simulink model "w3_warplab_trigger_proc"  (Simulink 7.7)
settings: Solver=ode45  StartTime=0.0  StopTime=60  RelTol=1e-3
InitFcn:
  | w3_warplab_trigger_proc_init
StartFcn:
  | w3_warplab_trigger_proc_init
undefined symbols (not defined in the file or in its folder): gcbh, xlBlockLoadCallback, xlGetNormalizedPeriod
libraries: xbsIndex_r4 x1289, xbsEDKLib_r4 x1, simulink x1
(part 3 of 10)

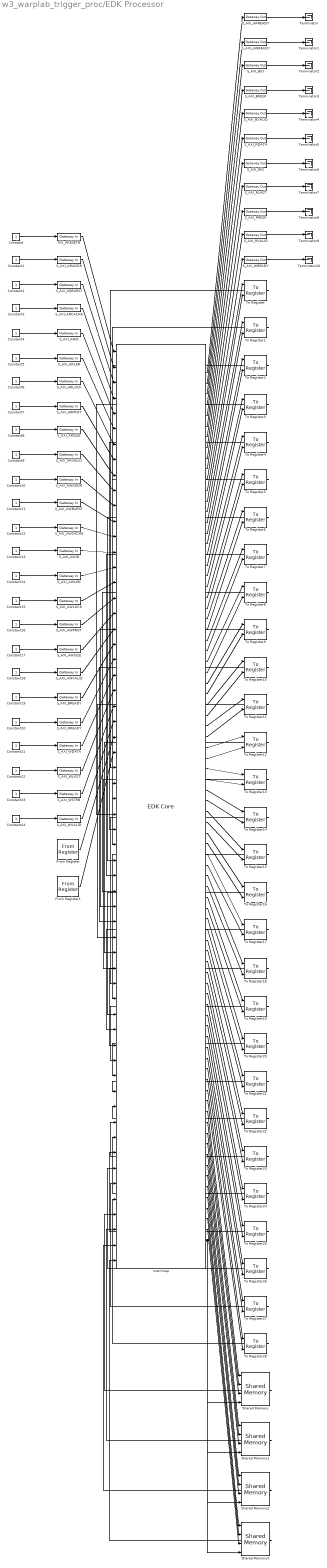
== system w3_warplab_trigger_proc/EDK Processor ==
  AXI_ARESETN : xbsIndex_r4/Gateway In  gui_display_data_type=Fixed-point  arith_type=Boolean  n_bits=16  bin_pt=14  preci_type=Single  exp_width=8  frac_width=24  quantization="Round  (unbiased: +/- Inf)"  overflow=Saturate  period=xlGetNormalizedPeriod()  dbl_ovrd=off  timing_constraint=None  locs_specified=off  LOCs={}  UseAsADC=off  ADCChannel='1'  inherit_from_input=off  hdl_port=on  block_type=gatewayin
  Constant{,1..24} (25 alike) : Constant
  From Register : xbsIndex_r4/From Register  shared_memory_name='CORE_INFO'  init=0  period=xlGetNormalizedPeriod()  ownership=Owned and initialized elsewhere  gui_display_data_type=Fixed-point  arith_type=Unsigned  n_bits=24  bin_pt=0  preci_type=Single  dbl_ovrd=off  block_type=fromreg
      settings: AttributesFormatString=<< %<shared_memory_name> >>  infoedit="Register block that reads data to a shared memory register.  Delay of one sample period."
  From Register1 : xbsIndex_r4/From Register  shared_memory_name='TRIG_OUT'  init=0  period=xlGetNormalizedPeriod()  ownership=Owned and initialized elsewhere  gui_display_data_type=Fixed-point  arith_type=Unsigned  n_bits=6  bin_pt=0  preci_type=Single  dbl_ovrd=off  block_type=fromreg
      settings: AttributesFormatString=<< %<shared_memory_name> >>  infoedit="Register block that reads data to a shared memory register.  Delay of one sample period."
  S_AXI_ARADDR : xbsIndex_r4/Gateway In  gui_display_data_type=Fixed-point  arith_type=Unsigned  n_bits=32  bin_pt=0  preci_type=Single  exp_width=8  frac_width=24  quantization="Round  (unbiased: +/- Inf)"  overflow=Saturate  period=xlGetNormalizedPeriod()  dbl_ovrd=off  timing_constraint=None  locs_specified=off  LOCs={}  UseAsADC=off  ADCChannel='1'  inherit_from_input=off  hdl_port=on  block_type=gatewayin
  S_AXI_ARBURST : xbsIndex_r4/Gateway In  gui_display_data_type=Fixed-point  arith_type=Unsigned  n_bits=2  bin_pt=0  preci_type=Single  exp_width=8  frac_width=24  quantization="Round  (unbiased: +/- Inf)"  overflow=Saturate  period=xlGetNormalizedPeriod()  dbl_ovrd=off  timing_constraint=None  locs_specified=off  LOCs={}  UseAsADC=off  ADCChannel='1'  inherit_from_input=off  hdl_port=on  block_type=gatewayin
  S_AXI_ARCACHE : xbsIndex_r4/Gateway In  gui_display_data_type=Fixed-point  arith_type=Unsigned  n_bits=4  bin_pt=0  preci_type=Single  exp_width=8  frac_width=24  quantization="Round  (unbiased: +/- Inf)"  overflow=Saturate  period=xlGetNormalizedPeriod()  dbl_ovrd=off  timing_constraint=None  locs_specified=off  LOCs={}  UseAsADC=off  ADCChannel='1'  inherit_from_input=off  hdl_port=on  block_type=gatewayin
  S_AXI_ARID : xbsIndex_r4/Gateway In  gui_display_data_type=Fixed-point  arith_type=Unsigned  n_bits=8  bin_pt=0  preci_type=Single  exp_width=8  frac_width=24  quantization="Round  (unbiased: +/- Inf)"  overflow=Saturate  period=xlGetNormalizedPeriod()  dbl_ovrd=off  timing_constraint=None  locs_specified=off  LOCs={}  UseAsADC=off  ADCChannel='1'  inherit_from_input=off  hdl_port=on  block_type=gatewayin
  S_AXI_ARLEN : xbsIndex_r4/Gateway In  gui_display_data_type=Fixed-point  arith_type=Unsigned  n_bits=8  bin_pt=0  preci_type=Single  exp_width=8  frac_width=24  quantization="Round  (unbiased: +/- Inf)"  overflow=Saturate  period=xlGetNormalizedPeriod()  dbl_ovrd=off  timing_constraint=None  locs_specified=off  LOCs={}  UseAsADC=off  ADCChannel='1'  inherit_from_input=off  hdl_port=on  block_type=gatewayin
  S_AXI_ARLOCK : xbsIndex_r4/Gateway In  gui_display_data_type=Fixed-point  arith_type=Unsigned  n_bits=2  bin_pt=0  preci_type=Single  exp_width=8  frac_width=24  quantization="Round  (unbiased: +/- Inf)"  overflow=Saturate  period=xlGetNormalizedPeriod()  dbl_ovrd=off  timing_constraint=None  locs_specified=off  LOCs={}  UseAsADC=off  ADCChannel='1'  inherit_from_input=off  hdl_port=on  block_type=gatewayin
  S_AXI_ARPROT : xbsIndex_r4/Gateway In  gui_display_data_type=Fixed-point  arith_type=Unsigned  n_bits=3  bin_pt=0  preci_type=Single  exp_width=8  frac_width=24  quantization="Round  (unbiased: +/- Inf)"  overflow=Saturate  period=xlGetNormalizedPeriod()  dbl_ovrd=off  timing_constraint=None  locs_specified=off  LOCs={}  UseAsADC=off  ADCChannel='1'  inherit_from_input=off  hdl_port=on  block_type=gatewayin
  S_AXI_ARREADY : xbsIndex_r4/Gateway Out  inherit_from_input=off  hdl_port=on  timing_constraint=None  locs_specified=off  LOCs={}  UseAsDAC=off  DACChannel='1'  block_type=gatewayout
  S_AXI_ARSIZE : xbsIndex_r4/Gateway In  gui_display_data_type=Fixed-point  arith_type=Unsigned  n_bits=3  bin_pt=0  preci_type=Single  exp_width=8  frac_width=24  quantization="Round  (unbiased: +/- Inf)"  overflow=Saturate  period=xlGetNormalizedPeriod()  dbl_ovrd=off  timing_constraint=None  locs_specified=off  LOCs={}  UseAsADC=off  ADCChannel='1'  inherit_from_input=off  hdl_port=on  block_type=gatewayin
  S_AXI_ARVALID : xbsIndex_r4/Gateway In  gui_display_data_type=Fixed-point  arith_type=Boolean  n_bits=16  bin_pt=14  preci_type=Single  exp_width=8  frac_width=24  quantization="Round  (unbiased: +/- Inf)"  overflow=Saturate  period=xlGetNormalizedPeriod()  dbl_ovrd=off  timing_constraint=None  locs_specified=off  LOCs={}  UseAsADC=off  ADCChannel='1'  inherit_from_input=off  hdl_port=on  block_type=gatewayin
  S_AXI_AWADDR : xbsIndex_r4/Gateway In  gui_display_data_type=Fixed-point  arith_type=Unsigned  n_bits=32  bin_pt=0  preci_type=Single  exp_width=8  frac_width=24  quantization="Round  (unbiased: +/- Inf)"  overflow=Saturate  period=xlGetNormalizedPeriod()  dbl_ovrd=off  timing_constraint=None  locs_specified=off  LOCs={}  UseAsADC=off  ADCChannel='1'  inherit_from_input=off  hdl_port=on  block_type=gatewayin
  S_AXI_AWBURST : xbsIndex_r4/Gateway In  gui_display_data_type=Fixed-point  arith_type=Unsigned  n_bits=2  bin_pt=0  preci_type=Single  exp_width=8  frac_width=24  quantization="Round  (unbiased: +/- Inf)"  overflow=Saturate  period=xlGetNormalizedPeriod()  dbl_ovrd=off  timing_constraint=None  locs_specified=off  LOCs={}  UseAsADC=off  ADCChannel='1'  inherit_from_input=off  hdl_port=on  block_type=gatewayin
  S_AXI_AWCACHE : xbsIndex_r4/Gateway In  gui_display_data_type=Fixed-point  arith_type=Unsigned  n_bits=4  bin_pt=0  preci_type=Single  exp_width=8  frac_width=24  quantization="Round  (unbiased: +/- Inf)"  overflow=Saturate  period=xlGetNormalizedPeriod()  dbl_ovrd=off  timing_constraint=None  locs_specified=off  LOCs={}  UseAsADC=off  ADCChannel='1'  inherit_from_input=off  hdl_port=on  block_type=gatewayin
  S_AXI_AWID : xbsIndex_r4/Gateway In  gui_display_data_type=Fixed-point  arith_type=Unsigned  n_bits=8  bin_pt=0  preci_type=Single  exp_width=8  frac_width=24  quantization="Round  (unbiased: +/- Inf)"  overflow=Saturate  period=xlGetNormalizedPeriod()  dbl_ovrd=off  timing_constraint=None  locs_specified=off  LOCs={}  UseAsADC=off  ADCChannel='1'  inherit_from_input=off  hdl_port=on  block_type=gatewayin
  S_AXI_AWLEN : xbsIndex_r4/Gateway In  gui_display_data_type=Fixed-point  arith_type=Unsigned  n_bits=8  bin_pt=0  preci_type=Single  exp_width=8  frac_width=24  quantization="Round  (unbiased: +/- Inf)"  overflow=Saturate  period=xlGetNormalizedPeriod()  dbl_ovrd=off  timing_constraint=None  locs_specified=off  LOCs={}  UseAsADC=off  ADCChannel='1'  inherit_from_input=off  hdl_port=on  block_type=gatewayin
  S_AXI_AWLOCK : xbsIndex_r4/Gateway In  gui_display_data_type=Fixed-point  arith_type=Unsigned  n_bits=2  bin_pt=0  preci_type=Single  exp_width=8  frac_width=24  quantization="Round  (unbiased: +/- Inf)"  overflow=Saturate  period=xlGetNormalizedPeriod()  dbl_ovrd=off  timing_constraint=None  locs_specified=off  LOCs={}  UseAsADC=off  ADCChannel='1'  inherit_from_input=off  hdl_port=on  block_type=gatewayin
  S_AXI_AWPROT : xbsIndex_r4/Gateway In  gui_display_data_type=Fixed-point  arith_type=Unsigned  n_bits=3  bin_pt=0  preci_type=Single  exp_width=8  frac_width=24  quantization="Round  (unbiased: +/- Inf)"  overflow=Saturate  period=xlGetNormalizedPeriod()  dbl_ovrd=off  timing_constraint=None  locs_specified=off  LOCs={}  UseAsADC=off  ADCChannel='1'  inherit_from_input=off  hdl_port=on  block_type=gatewayin
  S_AXI_AWREADY : xbsIndex_r4/Gateway Out  inherit_from_input=off  hdl_port=on  timing_constraint=None  locs_specified=off  LOCs={}  UseAsDAC=off  DACChannel='1'  block_type=gatewayout
  S_AXI_AWSIZE : xbsIndex_r4/Gateway In  gui_display_data_type=Fixed-point  arith_type=Unsigned  n_bits=3  bin_pt=0  preci_type=Single  exp_width=8  frac_width=24  quantization="Round  (unbiased: +/- Inf)"  overflow=Saturate  period=xlGetNormalizedPeriod()  dbl_ovrd=off  timing_constraint=None  locs_specified=off  LOCs={}  UseAsADC=off  ADCChannel='1'  inherit_from_input=off  hdl_port=on  block_type=gatewayin
  S_AXI_AWVALID : xbsIndex_r4/Gateway In  gui_display_data_type=Fixed-point  arith_type=Boolean  n_bits=16  bin_pt=14  preci_type=Single  exp_width=8  frac_width=24  quantization="Round  (unbiased: +/- Inf)"  overflow=Saturate  period=xlGetNormalizedPeriod()  dbl_ovrd=off  timing_constraint=None  locs_specified=off  LOCs={}  UseAsADC=off  ADCChannel='1'  inherit_from_input=off  hdl_port=on  block_type=gatewayin
  S_AXI_BID : xbsIndex_r4/Gateway Out  inherit_from_input=off  hdl_port=on  timing_constraint=None  locs_specified=off  LOCs={}  UseAsDAC=off  DACChannel='1'  block_type=gatewayout
  S_AXI_BREADY : xbsIndex_r4/Gateway In  gui_display_data_type=Fixed-point  arith_type=Boolean  n_bits=16  bin_pt=14  preci_type=Single  exp_width=8  frac_width=24  quantization="Round  (unbiased: +/- Inf)"  overflow=Saturate  period=xlGetNormalizedPeriod()  dbl_ovrd=off  timing_constraint=None  locs_specified=off  LOCs={}  UseAsADC=off  ADCChannel='1'  inherit_from_input=off  hdl_port=on  block_type=gatewayin
  S_AXI_BRESP : xbsIndex_r4/Gateway Out  inherit_from_input=off  hdl_port=on  timing_constraint=None  locs_specified=off  LOCs={}  UseAsDAC=off  DACChannel='1'  block_type=gatewayout
  S_AXI_BVALID : xbsIndex_r4/Gateway Out  inherit_from_input=off  hdl_port=on  timing_constraint=None  locs_specified=off  LOCs={}  UseAsDAC=off  DACChannel='1'  block_type=gatewayout
  S_AXI_RDATA : xbsIndex_r4/Gateway Out  inherit_from_input=off  hdl_port=on  timing_constraint=None  locs_specified=off  LOCs={}  UseAsDAC=off  DACChannel='1'  block_type=gatewayout
  S_AXI_RID : xbsIndex_r4/Gateway Out  inherit_from_input=off  hdl_port=on  timing_constraint=None  locs_specified=off  LOCs={}  UseAsDAC=off  DACChannel='1'  block_type=gatewayout
  S_AXI_RLAST : xbsIndex_r4/Gateway Out  inherit_from_input=off  hdl_port=on  timing_constraint=None  locs_specified=off  LOCs={}  UseAsDAC=off  DACChannel='1'  block_type=gatewayout
  S_AXI_RREADY : xbsIndex_r4/Gateway In  gui_display_data_type=Fixed-point  arith_type=Boolean  n_bits=16  bin_pt=14  preci_type=Single  exp_width=8  frac_width=24  quantization="Round  (unbiased: +/- Inf)"  overflow=Saturate  period=xlGetNormalizedPeriod()  dbl_ovrd=off  timing_constraint=None  locs_specified=off  LOCs={}  UseAsADC=off  ADCChannel='1'  inherit_from_input=off  hdl_port=on  block_type=gatewayin
  S_AXI_RRESP : xbsIndex_r4/Gateway Out  inherit_from_input=off  hdl_port=on  timing_constraint=None  locs_specified=off  LOCs={}  UseAsDAC=off  DACChannel='1'  block_type=gatewayout
  S_AXI_RVALID : xbsIndex_r4/Gateway Out  inherit_from_input=off  hdl_port=on  timing_constraint=None  locs_specified=off  LOCs={}  UseAsDAC=off  DACChannel='1'  block_type=gatewayout
  S_AXI_WDATA : xbsIndex_r4/Gateway In  gui_display_data_type=Fixed-point  arith_type=Unsigned  n_bits=32  bin_pt=0  preci_type=Single  exp_width=8  frac_width=24  quantization="Round  (unbiased: +/- Inf)"  overflow=Saturate  period=xlGetNormalizedPeriod()  dbl_ovrd=off  timing_constraint=None  locs_specified=off  LOCs={}  UseAsADC=off  ADCChannel='1'  inherit_from_input=off  hdl_port=on  block_type=gatewayin
  S_AXI_WLAST : xbsIndex_r4/Gateway In  gui_display_data_type=Fixed-point  arith_type=Boolean  n_bits=16  bin_pt=14  preci_type=Single  exp_width=8  frac_width=24  quantization="Round  (unbiased: +/- Inf)"  overflow=Saturate  period=xlGetNormalizedPeriod()  dbl_ovrd=off  timing_constraint=None  locs_specified=off  LOCs={}  UseAsADC=off  ADCChannel='1'  inherit_from_input=off  hdl_port=on  block_type=gatewayin
  S_AXI_WREADY : xbsIndex_r4/Gateway Out  inherit_from_input=off  hdl_port=on  timing_constraint=None  locs_specified=off  LOCs={}  UseAsDAC=off  DACChannel='1'  block_type=gatewayout
  S_AXI_WSTRB : xbsIndex_r4/Gateway In  gui_display_data_type=Fixed-point  arith_type=Unsigned  n_bits=4  bin_pt=0  preci_type=Single  exp_width=8  frac_width=24  quantization="Round  (unbiased: +/- Inf)"  overflow=Saturate  period=xlGetNormalizedPeriod()  dbl_ovrd=off  timing_constraint=None  locs_specified=off  LOCs={}  UseAsADC=off  ADCChannel='1'  inherit_from_input=off  hdl_port=on  block_type=gatewayin
  S_AXI_WVALID : xbsIndex_r4/Gateway In  gui_display_data_type=Fixed-point  arith_type=Boolean  n_bits=16  bin_pt=14  preci_type=Single  exp_width=8  frac_width=24  quantization="Round  (unbiased: +/- Inf)"  overflow=Saturate  period=xlGetNormalizedPeriod()  dbl_ovrd=off  timing_constraint=None  locs_specified=off  LOCs={}  UseAsADC=off  ADCChannel='1'  inherit_from_input=off  hdl_port=on  block_type=gatewayin
  Shared Memory : xbsIndex_r4/Shared Memory  shared_memory_name='PktOps1'  depth=64  ownership=Owned and Initialized Elsewhere  initVector=sin(pi*(0:15)/16)  en=on  mutex=Unprotected  mode=Read and Write  write_mode=Read Before Write  time_out=0  latency=1  explicit_data_type=off  gui_display_data_type=Fixed-point  arith_type=Unsigned  n_bits=32  bin_pt=0  preci_type=Single  implementation=Block RAM  use_rpm=off  block_type=shmem
      settings: AttributesFormatString=<< %<shared_memory_name> >>
  Shared Memory1 : xbsIndex_r4/Shared Memory  shared_memory_name='PktTemplate1'  depth=64  ownership=Owned and Initialized Elsewhere  initVector=sin(pi*(0:15)/16)  en=on  mutex=Unprotected  mode=Read and Write  write_mode=Read Before Write  time_out=0  latency=1  explicit_data_type=off  gui_display_data_type=Fixed-point  arith_type=Unsigned  n_bits=32  bin_pt=0  preci_type=Single  implementation=Block RAM  use_rpm=off  block_type=shmem
      settings: AttributesFormatString=<< %<shared_memory_name> >>
  Shared Memory2 : xbsIndex_r4/Shared Memory  shared_memory_name='PktOps0'  depth=64  ownership=Owned and Initialized Elsewhere  initVector=sin(pi*(0:15)/16)  en=on  mutex=Unprotected  mode=Read and Write  write_mode=Read Before Write  time_out=0  latency=1  explicit_data_type=off  gui_display_data_type=Fixed-point  arith_type=Unsigned  n_bits=32  bin_pt=0  preci_type=Single  implementation=Block RAM  use_rpm=off  block_type=shmem
      settings: AttributesFormatString=<< %<shared_memory_name> >>
  Shared Memory3 : xbsIndex_r4/Shared Memory  shared_memory_name='PktTemplate0'  depth=64  ownership=Owned and Initialized Elsewhere  initVector=sin(pi*(0:15)/16)  en=on  mutex=Unprotected  mode=Read and Write  write_mode=Read Before Write  time_out=0  latency=1  explicit_data_type=off  gui_display_data_type=Fixed-point  arith_type=Unsigned  n_bits=32  bin_pt=0  preci_type=Single  implementation=Block RAM  use_rpm=off  block_type=shmem
      settings: AttributesFormatString=<< %<shared_memory_name> >>
  Terminator{,1..10} (11 alike) : Terminator
  To Register : xbsIndex_r4/To Register  shared_memory_name='TRIG_ODELAY_CFG_CMPLL'  init=0  ownership=Owned and initialized elsewhere  explicit_data_type=on  gui_display_data_type=Fixed-point  arith_type=Unsigned  n_bits=32  bin_pt=0  preci_type=Single  dbl_ovrd=off  block_type=toreg
      settings: AttributesFormatString=<< %<shared_memory_name> >>  infoedit="Register block that writes data to a shared memory register.  Delay of one sample period."
  To Register1 : xbsIndex_r4/To Register  shared_memory_name='TRIG_IDELAY_CFG_CMPLL'  init=0  ownership=Owned and initialized elsewhere  explicit_data_type=on  gui_display_data_type=Fixed-point  arith_type=Unsigned  n_bits=32  bin_pt=0  preci_type=Single  dbl_ovrd=off  block_type=toreg
      settings: AttributesFormatString=<< %<shared_memory_name> >>  infoedit="Register block that writes data to a shared memory register.  Delay of one sample period."
  To Register10 : xbsIndex_r4/To Register  shared_memory_name='TRIG_IN_CONF_2'  init=0  ownership=Owned and initialized elsewhere  explicit_data_type=on  gui_display_data_type=Fixed-point  arith_type=Unsigned  n_bits=32  bin_pt=0  preci_type=Single  dbl_ovrd=off  block_type=toreg
      settings: AttributesFormatString=<< %<shared_memory_name> >>  infoedit="Register block that writes data to a shared memory register.  Delay of one sample period."
  To Register11 : xbsIndex_r4/To Register  shared_memory_name='TRIG_IN_CONF_0'  init=0  ownership=Owned and initialized elsewhere  explicit_data_type=on  gui_display_data_type=Fixed-point  arith_type=Unsigned  n_bits=32  bin_pt=0  preci_type=Single  dbl_ovrd=off  block_type=toreg
      settings: AttributesFormatString=<< %<shared_memory_name> >>  infoedit="Register block that writes data to a shared memory register.  Delay of one sample period."
  To Register12 : xbsIndex_r4/To Register  shared_memory_name='TRIG_IN_CONF_8'  init=0  ownership=Owned and initialized elsewhere  explicit_data_type=on  gui_display_data_type=Fixed-point  arith_type=Unsigned  n_bits=32  bin_pt=0  preci_type=Single  dbl_ovrd=off  block_type=toreg
      settings: AttributesFormatString=<< %<shared_memory_name> >>  infoedit="Register block that writes data to a shared memory register.  Delay of one sample period."
  To Register13 : xbsIndex_r4/To Register  shared_memory_name='TRIG_IN_CONF_7'  init=0  ownership=Owned and initialized elsewhere  explicit_data_type=on  gui_display_data_type=Fixed-point  arith_type=Unsigned  n_bits=32  bin_pt=0  preci_type=Single  dbl_ovrd=off  block_type=toreg
      settings: AttributesFormatString=<< %<shared_memory_name> >>  infoedit="Register block that writes data to a shared memory register.  Delay of one sample period."
  To Register14 : xbsIndex_r4/To Register  shared_memory_name='TRIG_OUT_5_CONF_0'  init=0  ownership=Owned and initialized elsewhere  explicit_data_type=on  gui_display_data_type=Fixed-point  arith_type=Unsigned  n_bits=32  bin_pt=0  preci_type=Single  dbl_ovrd=off  block_type=toreg
      settings: AttributesFormatString=<< %<shared_memory_name> >>  infoedit="Register block that writes data to a shared memory register.  Delay of one sample period."
  To Register15 : xbsIndex_r4/To Register  shared_memory_name='TRIG_OUT_5_CONF_1'  init=0  ownership=Owned and initialized elsewhere  explicit_data_type=on  gui_display_data_type=Fixed-point  arith_type=Unsigned  n_bits=32  bin_pt=0  preci_type=Single  dbl_ovrd=off  block_type=toreg
      settings: AttributesFormatString=<< %<shared_memory_name> >>  infoedit="Register block that writes data to a shared memory register.  Delay of one sample period."
  To Register16 : xbsIndex_r4/To Register  shared_memory_name='TRIG_OUT_4_CONF_0'  init=0  ownership=Owned and initialized elsewhere  explicit_data_type=on  gui_display_data_type=Fixed-point  arith_type=Unsigned  n_bits=32  bin_pt=0  preci_type=Single  dbl_ovrd=off  block_type=toreg
      settings: AttributesFormatString=<< %<shared_memory_name> >>  infoedit="Register block that writes data to a shared memory register.  Delay of one sample period."
  To Register17 : xbsIndex_r4/To Register  shared_memory_name='TRIG_OUT_0_CONF_0'  init=0  ownership=Owned and initialized elsewhere  explicit_data_type=on  gui_display_data_type=Fixed-point  arith_type=Unsigned  n_bits=32  bin_pt=0  preci_type=Single  dbl_ovrd=off  block_type=toreg
      settings: AttributesFormatString=<< %<shared_memory_name> >>  infoedit="Register block that writes data to a shared memory register.  Delay of one sample period."
  To Register18 : xbsIndex_r4/To Register  shared_memory_name='TRIG_OUT_4_CONF_1'  init=0  ownership=Owned and initialized elsewhere  explicit_data_type=on  gui_display_data_type=Fixed-point  arith_type=Unsigned  n_bits=32  bin_pt=0  preci_type=Single  dbl_ovrd=off  block_type=toreg
      settings: AttributesFormatString=<< %<shared_memory_name> >>  infoedit="Register block that writes data to a shared memory register.  Delay of one sample period."
  To Register19 : xbsIndex_r4/To Register  shared_memory_name='TRIG_OUT_3_CONF_0'  init=0  ownership=Owned and initialized elsewhere  explicit_data_type=on  gui_display_data_type=Fixed-point  arith_type=Unsigned  n_bits=32  bin_pt=0  preci_type=Single  dbl_ovrd=off  block_type=toreg
      settings: AttributesFormatString=<< %<shared_memory_name> >>  infoedit="Register block that writes data to a shared memory register.  Delay of one sample period."
  To Register2 : xbsIndex_r4/To Register  shared_memory_name='TRIG_ODELAY_CFG_DEBUG_HDR'  init=0  ownership=Owned and initialized elsewhere  explicit_data_type=on  gui_display_data_type=Fixed-point  arith_type=Unsigned  n_bits=32  bin_pt=0  preci_type=Single  dbl_ovrd=off  block_type=toreg
      settings: AttributesFormatString=<< %<shared_memory_name> >>  infoedit="Register block that writes data to a shared memory register.  Delay of one sample period."
  To Register20 : xbsIndex_r4/To Register  shared_memory_name='TRIG_OUT_3_CONF_1'  init=0  ownership=Owned and initialized elsewhere  explicit_data_type=on  gui_display_data_type=Fixed-point  arith_type=Unsigned  n_bits=32  bin_pt=0  preci_type=Single  dbl_ovrd=off  block_type=toreg
      settings: AttributesFormatString=<< %<shared_memory_name> >>  infoedit="Register block that writes data to a shared memory register.  Delay of one sample period."
  To Register21 : xbsIndex_r4/To Register  shared_memory_name='TRIG_OUT_2_CONF_0'  init=0  ownership=Owned and initialized elsewhere  explicit_data_type=on  gui_display_data_type=Fixed-point  arith_type=Unsigned  n_bits=32  bin_pt=0  preci_type=Single  dbl_ovrd=off  block_type=toreg
      settings: AttributesFormatString=<< %<shared_memory_name> >>  infoedit="Register block that writes data to a shared memory register.  Delay of one sample period."
  To Register22 : xbsIndex_r4/To Register  shared_memory_name='TRIG_OUT_2_CONF_1'  init=0  ownership=Owned and initialized elsewhere  explicit_data_type=on  gui_display_data_type=Fixed-point  arith_type=Unsigned  n_bits=32  bin_pt=0  preci_type=Single  dbl_ovrd=off  block_type=toreg
      settings: AttributesFormatString=<< %<shared_memory_name> >>  infoedit="Register block that writes data to a shared memory register.  Delay of one sample period."
  To Register23 : xbsIndex_r4/To Register  shared_memory_name='TRIG_OUT_1_CONF_0'  init=0  ownership=Owned and initialized elsewhere  explicit_data_type=on  gui_display_data_type=Fixed-point  arith_type=Unsigned  n_bits=32  bin_pt=0  preci_type=Single  dbl_ovrd=off  block_type=toreg
      settings: AttributesFormatString=<< %<shared_memory_name> >>  infoedit="Register block that writes data to a shared memory register.  Delay of one sample period."
  To Register24 : xbsIndex_r4/To Register  shared_memory_name='TRIG_OUT_1_CONF_1'  init=0  ownership=Owned and initialized elsewhere  explicit_data_type=on  gui_display_data_type=Fixed-point  arith_type=Unsigned  n_bits=32  bin_pt=0  preci_type=Single  dbl_ovrd=off  block_type=toreg
      settings: AttributesFormatString=<< %<shared_memory_name> >>  infoedit="Register block that writes data to a shared memory register.  Delay of one sample period."
  To Register25 : xbsIndex_r4/To Register  shared_memory_name='TRIG_OUT_0_CONF_1'  init=0  ownership=Owned and initialized elsewhere  explicit_data_type=on  gui_display_data_type=Fixed-point  arith_type=Unsigned  n_bits=32  bin_pt=0  preci_type=Single  dbl_ovrd=off  block_type=toreg
      settings: AttributesFormatString=<< %<shared_memory_name> >>  infoedit="Register block that writes data to a shared memory register.  Delay of one sample period."
  To Register26 : xbsIndex_r4/To Register  shared_memory_name='RSSI_PKT_DET_DURATIONS'  init=0  ownership=Owned and initialized elsewhere  explicit_data_type=on  gui_display_data_type=Fixed-point  arith_type=Unsigned  n_bits=32  bin_pt=0  preci_type=Single  dbl_ovrd=off  block_type=toreg
      settings: AttributesFormatString=<< %<shared_memory_name> >>  infoedit="Register block that writes data to a shared memory register.  Delay of one sample period."
  To Register27 : xbsIndex_r4/To Register  shared_memory_name='RSSI_PKT_DET_THRESHOLDS'  init=0  ownership=Owned and initialized elsewhere  explicit_data_type=on  gui_display_data_type=Fixed-point  arith_type=Unsigned  n_bits=32  bin_pt=0  preci_type=Single  dbl_ovrd=off  block_type=toreg
      settings: AttributesFormatString=<< %<shared_memory_name> >>  infoedit="Register block that writes data to a shared memory register.  Delay of one sample period."
  To Register28 : xbsIndex_r4/To Register  shared_memory_name='TRIG_IN_CONF_1'  init=0  ownership=Owned and initialized elsewhere  explicit_data_type=on  gui_display_data_type=Fixed-point  arith_type=Unsigned  n_bits=32  bin_pt=0  preci_type=Single  dbl_ovrd=off  block_type=toreg
      settings: AttributesFormatString=<< %<shared_memory_name> >>  infoedit="Register block that writes data to a shared memory register.  Delay of one sample period."
  To Register3 : xbsIndex_r4/To Register  shared_memory_name='TRIG_IDELAY_CFG_DEBUG_HDR'  init=0  ownership=Owned and initialized elsewhere  explicit_data_type=on  gui_display_data_type=Fixed-point  arith_type=Unsigned  n_bits=32  bin_pt=0  preci_type=Single  dbl_ovrd=off  block_type=toreg
      settings: AttributesFormatString=<< %<shared_memory_name> >>  infoedit="Register block that writes data to a shared memory register.  Delay of one sample period."
  To Register4 : xbsIndex_r4/To Register  shared_memory_name='TRIG_IODELAYS_CONTROL'  init=0  ownership=Owned and initialized elsewhere  explicit_data_type=on  gui_display_data_type=Fixed-point  arith_type=Unsigned  n_bits=32  bin_pt=0  preci_type=Single  dbl_ovrd=off  block_type=toreg
      settings: AttributesFormatString=<< %<shared_memory_name> >>  infoedit="Register block that writes data to a shared memory register.  Delay of one sample period."
  To Register5 : xbsIndex_r4/To Register  shared_memory_name='RSSI_PKT_DET_CONFIG'  init=0  ownership=Owned and initialized elsewhere  explicit_data_type=on  gui_display_data_type=Fixed-point  arith_type=Unsigned  n_bits=32  bin_pt=0  preci_type=Single  dbl_ovrd=off  block_type=toreg
      settings: AttributesFormatString=<< %<shared_memory_name> >>  infoedit="Register block that writes data to a shared memory register.  Delay of one sample period."
  To Register6 : xbsIndex_r4/To Register  shared_memory_name='TRIG_IN_CONF_6'  init=0  ownership=Owned and initialized elsewhere  explicit_data_type=on  gui_display_data_type=Fixed-point  arith_type=Unsigned  n_bits=32  bin_pt=0  preci_type=Single  dbl_ovrd=off  block_type=toreg
      settings: AttributesFormatString=<< %<shared_memory_name> >>  infoedit="Register block that writes data to a shared memory register.  Delay of one sample period."
  To Register7 : xbsIndex_r4/To Register  shared_memory_name='TRIG_IN_CONF_5'  init=0  ownership=Owned and initialized elsewhere  explicit_data_type=on  gui_display_data_type=Fixed-point  arith_type=Unsigned  n_bits=32  bin_pt=0  preci_type=Single  dbl_ovrd=off  block_type=toreg
      settings: AttributesFormatString=<< %<shared_memory_name> >>  infoedit="Register block that writes data to a shared memory register.  Delay of one sample period."
  To Register8 : xbsIndex_r4/To Register  shared_memory_name='TRIG_IN_CONF_4'  init=0  ownership=Owned and initialized elsewhere  explicit_data_type=on  gui_display_data_type=Fixed-point  arith_type=Unsigned  n_bits=32  bin_pt=0  preci_type=Single  dbl_ovrd=off  block_type=toreg
      settings: AttributesFormatString=<< %<shared_memory_name> >>  infoedit="Register block that writes data to a shared memory register.  Delay of one sample period."
  To Register9 : xbsIndex_r4/To Register  shared_memory_name='TRIG_IN_CONF_3'  init=0  ownership=Owned and initialized elsewhere  explicit_data_type=on  gui_display_data_type=Fixed-point  arith_type=Unsigned  n_bits=32  bin_pt=0  preci_type=Single  dbl_ovrd=off  block_type=toreg
      settings: AttributesFormatString=<< %<shared_memory_name> >>  infoedit="Register block that writes data to a shared memory register.  Delay of one sample period."
  memmap : xbsEDKLib_r4/EDK Core  sim_method=Inactive  xmp=xmp  blockname=blockname  dual_clock=dual_clock  procinfo=procinfo  bus_type=bus_type  memxtable=memxtable  memmap_hdlcontent=|  config={'inports'=>[{'arith_type'=>2.00000000000000000,'bin_pt'=>0.00000000000000000,'name'=>'AXI_ARESETN','width'=>0},{'arith_type'=>2.00000000000000000,'bin_pt'=>0.00000000000000000,'name'=>'S_AXI_ARADDR','width'=>32},{'arith_type'=>2.00000000000000000,'bin_pt'=>0.00000000000000000,'name'=>'S_AXI_ARBURST','width'=>2},{'arith_type'=>2.00000000000000000,'bin_pt'=>0.00000000000000000,'name'=>'S_AXI_ARCACHE','width'=>4},{'arith_type'=>2.00000000000000000,'bin_pt'=>0.00000000000000000,'name'=>'S_AXI_ARID','width'=>8},{'arith_type'=>2.00000000000000000,'bin_pt'=>0.00000000000000000,'name'=>'S_AXI_ARLEN','width'=>8},{'arith_type'=>2.00000000000000000,'bin_pt'=>0.00000000000000000,'name'=>'S_AXI_ARLOCK','width'=>2},{'arith_type'=>2.00000000000000000,'bin_pt'=>0.00000000000000000,'name'=>'S_AXI_ARPROT','width'=>3},{'arith_type'=>2.00000000000000000,'bin_pt'=>0.00000000000000000,'name'=>'S_AXI_ARSIZE','width'=>3},{'arith_type'=>2.00000000000000000,'bin_pt'=>0.00000000000000000,'name'=>'S_AXI_ARVALID','width'=>0},{'arith_type'=>2.00000000000000000,'bin_pt'=>0.00000000000000000,'name'=>'S_AXI_AWADDR','width'=>32},{'arith_type'=>2.00000000000000000,'bin_pt'=>0.00000000000000000,'name'=>'S_AXI_AWBURST','width'=>2},{'arith_type'=>2.00000000000000000,'bin_pt'=>0.00000000000000000,'name'=>'S_AXI_AWCACHE','width'=>4},{'arith_type'=>2.00000000000000000,'bin_pt'=>0.00000000000000000,'name'=>'S_AXI_AWID','width'=>8},{'arith_type'=>2.00000000000000000,'bin_pt'=>0.00000000000000000,'name'=>'S_AXI_AWLEN','width'=>8},{'arith_type'=>2.00000000000000000,'bin_pt'=>0.00000000000000000,'name'=>'S_AXI_AWLOCK','width'=>2},{'arith_type'=>2.00000000000000000,'bin_pt'=>0.00000000000000000,'name'=>'S_AXI_AWPROT','width'=>3},{'arith_type'=>2.00000000000000000,'bin_pt'=>0.00000000000000000,'name'=>'S_AXI_AWSIZE','width'=>3},{'arith_type'=>2.00000000000000000,'bin_pt'=>0.00000000000000000,'name'=>'S_AXI_AWVALID','width'=>0},{'arith_type'=>2.00000000000000000,'bin_pt'=>0.00000000000000000,'name'=>'S_AXI_BREADY','width'=>0},{'arith_type'=>2.00000000000000000,'bin_pt'=>0.00000000000000000,'name'=>'S_AXI_RREADY','width'=>0},{'arith_type'=>2.00000000000000000,'bin_pt'=>0.00000000000000000,'name'=>'S_AXI_WDATA','width'=>32},{'arith_type'=>2.00000000000000000,'bin_pt'=>0.00000000000000000,'name'=>'S_AXI_WLAST','width'=>0},{'arith_type'=>2.00000000000000000,'bin_pt'=>0.00000000000000000,'name'=>'S_AXI_WSTRB','width'=>4},{'arith_type'=>2.00000000000000000,'bin_pt'=>0.00000000000000000,'name'=>'S_AXI_WVALID','width'=>0},{'arith_type'=>2,'bin_pt'=>0,'name'=>'sm_CORE_INFO_dout','width'=>24},{'arith_type'=>2,'bin_pt'=>0,'name'=>'sm_TRIG_OUT_dout','width'=>6},{'arith_type'=>2,'bin_pt'=>0,'name'=>'sm_TRIG_ODELAY_CFG_CMPLL_dout','width'=>32},{'arith_type'=>2,'bin_pt'=>0,'name'=>'sm_TRIG_IDELAY_CFG_CMPLL_dout','width'=>32},{'arith_type'=>2,'bin_pt'=>0,'name'=>'sm_TRIG_ODELAY_CFG_DEBUG_HDR_dout','width'=>32},{'arith_type'=>2,'bin_pt'=>0,'name'=>'sm_TRIG_IDELAY_CFG_DEBUG_HDR_dout','width'=>32},{'arith_type'=>2,'bin_pt'=>0,'name'=>'sm_TRIG_IODELAYS_CONTROL_dout','width'=>32},{'arith_type'=>2,'bin_pt'=>0,'name'=>'sm_RSSI_PKT_DET_CONFIG_dout','width'=>32},{'arith_type'=>2,'bin_pt'=>0,'name'=>'sm_TRIG_IN_CONF_6_dout','width'=>32},{'arith_type'=>2,'bin_pt'=>0,'name'=>'sm_TRIG_IN_CONF_5_dout','width'=>32},{'arith_type'=>2,'bin_pt'=>0,'name'=>'sm_TRIG_IN_CONF_4_dout','width'=>32},{'arith_type'=>2,'bin_pt'=>0,'name'=>'sm_TRIG_IN_CONF_3_dout','width'=>32},{'arith_type'=>2,'bin_pt'=>0,'name'=>'sm_TRIG_IN_CONF_2_dout','width'=>32},{'arith_type'=>2,'bin_pt'=>0,'name'=>'sm_TRIG_IN_CONF_0_dout','width'=>32},{'arith_type'=>2,'bin_pt'=>0,'name'=>'sm_TRIG_IN_CONF_8_dout','width'=>32},{'arith_type'=>2,'bin_pt'=>0,'name'=>'sm_TRIG_IN_CONF_7_dout','width'=>32},{'arith_type'=>2,'bin_pt'=>0,'name'=>'sm_TRIG_OUT_5_CONF_0_dout','width'=>32},{'arith_type'=>2,'bin_pt'=>0,'name'=>'sm_TRIG_OUT_5_CONF_1_dout','width'=>32},{'arith_type'=>2,'bin_pt'=>0,'name'=>'sm_TRIG_OUT_4_CONF_0_dout','width'=>32},{'arith_type'=>2,'bin_pt'=>0,'name'=>'sm_TRIG_OUT_0_CONF_0_dout','width'=>32},{'arith_type'=>2,'bin_pt'=>0,'name'=>'sm_TRIG_OUT_4_CONF_1_dout','width'=>32},{'arith_type'=>2,'bin_pt'=>0,'name'=>'sm_TRIG_OUT_3_CONF_0_dout','width'=>32},{'arith_type'=>2,'bin_pt'=>0,'name'=>'sm_TRIG_OUT_3_CONF_1_dout','width'=>32},{'arith_type'=>2,'bin_pt'=>0,'name'=>'sm_TRIG_OUT_2_CONF_0_dout','width'=>32},{'arith_type'=>2,'bin_pt'=>0,'name'=>'sm_TRIG_OUT_2_CONF_1_dout','width'=>32},{'arith_type'=>2,'bin_pt'=>0,'name'=>'sm_TRIG_OUT_1_CONF_0_dout','width'=>32},{'arith_type'=>2,'bin_pt'=>0,'name'=>'sm_TRIG_OUT_1_CONF_1_dout','width'=>32},{'arith_type'=>2,'bin_pt'=>0,'name'=>'sm_TRIG_OUT_0_CONF_1_dout','width'=>32},{'arith_type'=>2,'bin_pt'=>0,'name'=>'sm_RSSI_PKT_DET_DURATIONS_dout','width'=>32},{'arith_type'=>2,'bin_pt'=>0,'name'=>'sm_RSSI_PKT_DET_THRESHOLDS_dout','width'=>32},{'arith_type'=>2,'bin_pt'=>0,'name'=>'sm_TRIG_IN_CONF_1_dout','width'=>32},{'arith_type'=>2,'bin_pt'=>0,'name'=>'sm_PktOps1_dout','width'=>32},{'arith_type'=>2,'bin_pt'=>0,'name'=>'sm_PktTemplate1_dout','width'=>32},{'arith_type'=>2,'bin_pt'=>0,'name'=>'sm_PktOps0_dout','width'=>32},{'arith_type'=>2,'bin_pt'=>0,'name'=>'sm_PktTemplate0_dout','width'=>32}],'outports'=>[{'arith_type'=>2.00000000000000000,'bin_pt'=>0.00000000000000000,'name'=>'S_AXI_ARREADY','width'=>0},{'arith_type'=>2.00000000000000000,'bin_pt'=>0.00000000000000000,'name'=>'S_AXI_AWREADY','width'=>0},{'arith_type'=>2.00000000000000000,'bin_pt'=>0.00000000000000000,'name'=>'S_AXI_BID','width'=>8},{'arith_type'=>2.00000000000000000,'bin_pt'=>0.00000000000000000,'name'=>'S_AXI_BRESP','width'=>2},{'arith_type'=>2.00000000000000000,'bin_pt'=>0.00000000000000000,'name'=>'S_AXI_BVALID','width'=>0},{'arith_type'=>2.00000000000000000,'bin_pt'=>0.00000000000000000,'name'=>'S_AXI_RDATA','width'=>32},{'arith_type'=>2.00000000000000000,'bin_pt'=>0.00000000000000000,'name'=>'S_AXI_RID','width'=>8},{'arith_type'=>2.00000000000000000,'bin_pt'=>0.00000000000000000,'name'=>'S_AXI_RLAST','width'=>0},{'arith_type'=>2.00000000000000000,'bin_pt'=>0.00000000000000000,'name'=>'S_AXI_RRESP','width'=>2},{'arith_type'=>2.00000000000000000,'bin_pt'=>0.00000000000000000,'name'=>'S_AXI_RVALID','width'=>0},{'arith_type'=>2.00000000000000000,'bin_pt'=>0.00000000000000000,'name'=>'S_AXI_WREADY','width'=>0},{'arith_type'=>2,'bin_pt'=>0,'name'=>'sm_TRIG_ODELAY_CFG_CMPLL_din','width'=>32},{'arith_type'=>2.00000000000000000,'bin_pt'=>0.00000000000000000,'name'=>'sm_TRIG_ODELAY_CFG_CMPLL_en','width'=>0.00000000000000000},{'arith_type'=>2,'bin_pt'=>0,'name'=>'sm_TRIG_IDELAY_CFG_CMPLL_din','width'=>32},{'arith_type'=>2.00000000000000000,'bin_pt'=>0.00000000000000000,'name'=>'sm_TRIG_IDELAY_CFG_CMPLL_en','width'=>0.00000000000000000},{'arith_type'=>2,'bin_pt'=>0,'name'=>'sm_TRIG_ODELAY_CFG_DEBUG_HDR_din','width'=>32},{'arith_type'=>2.00000000000000000,'bin_pt'=>0.00000000000000000,'name'=>'sm_TRIG_ODELAY_CFG_DEBUG_HDR_en','width'=>0.00000000000000000},{'arith_type'=>2,'bin_pt'=>0,'name'=>'sm_TRIG_IDELAY_CFG_DEBUG_HDR_din','width'=>32},{'arith_type'=>2.00000000000000000,'bin_pt'=>0.00000000000000000,'name'=>'sm_TRIG_IDELAY_CFG_DEBUG_HDR_en','width'=>0.00000000000000000},{'arith_type'=>2,'bin_pt'=>0,'name'=>'sm_TRIG_IODELAYS_CONTROL_din','width'=>32},{'arith_type'=>2.00000000000000000,'bin_pt'=>0.00000000000000000,'name'=>'sm_TRIG_IODELAYS_CONTROL_en','width'=>0.00000000000000000},{'arith_type'=>2,'bin_pt'=>0,'name'=>'sm_RSSI_PKT_DET_CONFIG_din','width'=>32},{'arith_type'=>2.00000000000000000,'bin_pt'=>0.00000000000000000,'name'=>'sm_RSSI_PKT_DET_CONFIG_en','width'=>0.00000000000000000},{'arith_type'=>2,'bin_pt'=>0,'name'=>'sm_TRIG_IN_CONF_6_din','width'=>32},{'arith_type'=>2.00000000000000000,'bin_pt'=>0.00000000000000000,'name'=>'sm_TRIG_IN_CONF_6_en','width'=>0.00000000000000000},{'arith_type'=>2,'bin_pt'=>0,'name'=>'sm_TRIG_IN_CONF_5_din','width'=>32},{'arith_type'=>2.00000000000000000,'bin_pt'=>0.00000000000000000,'name'=>'sm_TRIG_IN_CONF_5_en','width'=>0.00000000000000000},{'arith_type'=>2,'bin_pt'=>0,'name'=>'sm_TRIG_IN_CONF_4_din','width'=>32},{'arith_type'=>2.00000000000000000,'bin_pt'=>0.00000000000000000,'name'=>'sm_TRIG_IN_CONF_4_en','width'=>0.00000000000000000},{'arith_type'=>2,'bin_pt'=>0,'name'=>'sm_TRIG_IN_CONF_3_din','width'=>32},{'arith_type'=>2.00000000000000000,'bin_pt'=>0.00000000000000000,'name'=>'sm_TRIG_IN_CONF_3_en','width'=>0.00000000000000000},{'arith_type'=>2,'bin_pt'=>0,'name'=>'sm_TRIG_IN_CONF_2_din','width'=>32},{'arith_type'=>2.00000000000000000,'bin_pt'=>0.00000000000000000,'name'=>'sm_TRIG_IN_CONF_2_en','width'=>0.00000000000000000},{'arith_type'=>2,'bin_pt'=>0,'name'=>'sm_TRIG_IN_CONF_0_din','width'=>32},{'arith_type'=>2.00000000000000000,'bin_pt'=>0.00000000000000000,'name'=>'sm_TRIG_IN_CONF_0_en','width'=>0.00000000000000000},{'arith_type'=>2,'bin_pt'=>0,'name'=>'sm_TRIG_IN_CONF_8_din','width'=>32},{'arith_type'=>2.00000000000000000,'bin_pt'=>0.00000000000000000,'name'=>'sm_TRIG_IN_CONF_8_en','width'=>0.00000000000000000},{'arith_type'=>2,'bin_pt'=>0,'name'=>'sm_TRIG_IN_CONF_7_din','width'=>32},{'arith_type'=>2.00000000000000000,'bin_pt'=>0.00000000000000000,'name'=>'sm_TRIG_IN_CONF_7_en','width'=>0.00000000000000000},{'arith_type'=>2,'bin_pt'=>0,'name'=>'sm_TRIG_OUT_5_CONF_0_din','width'=>32},{'arith_type'=>2.00000000000000000,'bin_pt'=>0.00000000000000000,'name'=>'sm_TRIG_OUT_5_CONF_0_en','width'=>0.00000000000000000},{'arith_type'=>2,'bin_pt'=>0,'name'=>'sm_TRIG_OUT_5_CONF_1_din','width'=>32},{'arith_type'=>2.00000000000000000,'bin_pt'=>0.00000000000000000,'name'=>'sm_TRIG_OUT_5_CONF_1_en','width'=>0.00000000000000000},{'arith_type'=>2,'bin_pt'=>0,'name'=>'sm_TRIG_OUT_4_CONF_0_din','width'=>32},{'arith_type'=>2.00000000000000000,'bin_pt'=>0.00000000000000000,'name'=>'sm_TRIG_OUT_4_CONF_0_en','width'=>0.00000000000000000},{'arith_type'=>2,'bin_pt'=>0,'name'=>'sm_TRIG_OUT_0_CONF_0_din','width'=>32},{'arith_type'=>2.00000000000000000,'bin_pt'=>0.00000000000000000,'name'=>'sm_TRIG_OUT_0_CONF_0_en','width'=>0.00000000000000000},{'arith_type'=>2,'bin_pt'=>0,'name'=>'sm_TRIG_OUT_4_CONF_1_din','width'=>32},{'arith_type'=>2.00000000000000000,'bin_pt'=>0.00000000000000000,'name'=>'sm_TRIG_OUT_4_CONF_1_en','width'=>0.00000000000000000},{'arith_type'=>2,'bin_pt'=>0,'name'=>'sm_TRIG_OUT_3_CONF_0_din','width'=>32},{'arith_type'=>2.00000000000000000,'bin_pt'=>0.00000000000000000,'name'=>'sm_TRIG_OUT_3_CONF_0_en','width'=>0.00000000000000000},{'arith_type'=>2,'bin_pt'=>0,'name'=>'sm_TRIG_OUT_3_CONF_1_din','width'=>32},{'arith_type'=>2.00000000000000000,'bin_pt'=>0.00000000000000000,'name'=>'sm_TRIG_OUT_3_CONF_1_en','width'=>0.00000000000000000},{'arith_type'=>2,'bin_pt'=>0,'name'=>'sm_TRIG_OUT_2_CONF_0_din','width'=>32},{'arith_type'=>2.00000000000000000,'bin_pt'=>0.00000000000000000,'name'=>'sm_TRIG_OUT_2_CONF_0_en','width'=>0.00000000000000000},{'arith_type'=>2,'bin_pt'=>0,'name'=>'sm_TRIG_OUT_2_CONF_1_din','width'=>32},{'arith_type'=>2.00000000000000000,'bin_pt'=>0.00000000000000000,'name'=>'sm_TRIG_OUT_2_CONF_1_en','width'=>0.00000000000000000},{'arith_type'=>2,'bin_pt'=>0,'name'=>'sm_TRIG_OUT_1_CONF_0_din','width'=>32},{'arith_type'=>2.00000000000000000,'bin_pt'=>0.00000000000000000,'name'=>'sm_TRIG_OUT_1_CONF_0_en','width'=>0.00000000000000000},{'arith_type'=>2,'bin_pt'=>0,'name'=>'sm_TRIG_OUT_1_CONF_1_din','width'=>32},{'arith_type'=>2.00000000000000000,'bin_pt'=>0.00000000000000000,'name'=>'sm_TRIG_OUT_1_CONF_1_en','width'=>0.00000000000000000},{'arith_type'=>2,'bin_pt'=>0,'name'=>'sm_TRIG_OUT_0_CONF_1_din','width'=>32},{'arith_type'=>2.00000000000000000,'bin_pt'=>0.00000000000000000,'name'=>'sm_TRIG_OUT_0_CONF_1_en','width'=>0.00000000000000000},{'arith_type'=>2,'bin_pt'=>0,'name'=>'sm_RSSI_PKT_DET_DURATIONS_din','width'=>32},{'arith_type'=>2.00000000000000000,'bin_pt'=>0.00000000000000000,'name'=>'sm_RSSI_PKT_DET_DURATIONS_en','width'=>0.00000000000000000},{'arith_type'=>2,'bin_pt'=>0,'name'=>'sm_RSSI_PKT_DET_THRESHOLDS_din','width'=>32},{'arith_type'=>2.00000000000000000,'bin_pt'=>0.00000000000000000,'name'=>'sm_RSSI_PKT_DET_THRESHOLDS_en','width'=>0.00000000000000000},{'arith_type'=>2,'bin_pt'=>0,'name'=>'sm_TRIG_IN_CONF_1_din','width'=>32},{'arith_type'=>2.00000000000000000,'bin_pt'=>0.00000000000000000,'name'=>'sm_TRIG_IN_CONF_1_en','width'=>0.00000000000000000},{'arith_type'=>2.00000000000000000,'bin_pt'=>0.00000000000000000,'name'=>'sm_PktOps1_addr','width'=>6.00000000000000000},{'arith_type'=>2,'bin_pt'=>0,'name'=>'sm_PktOps1_din','width'=>32},{'arith_type'=>2.00000000000000000,'bin_pt'=>0.00000000000000000,'name'=>'sm_PktOps1_we','width'=>0.00000000000000000},{'arith_type'=>2.00000000000000000,'bin_pt'=>0.00000000000000000,'name'=>'sm_PktTemplate1_addr','width'=>6.00000000000000000},{'arith_type'=>2,'bin_pt'=>0,'name'=>'sm_PktTemplate1_din','width'=>32},{'arith_type'=>2.00000000000000000,'bin_pt'=>0.00000000000000000,'name'=>'sm_PktTemplate1_we','width'=>0.00000000000000000},{'arith_type'=>2.00000000000000000,'bin_pt'=>0.00000000000000000,'name'=>'sm_PktOps0_addr','width'=>6.00000000000000000},{'arith_type'=>2,'bin_pt'=>0,'name'=>'sm_PktOps0_din','width'=>32},{'arith_type'=>2.00000000000000000,'bin_pt'=>0.00000000000000000,'name'=>'sm_PktOps0_we','width'=>0.00000000000000000},{'arith_type'=>2.00000000000000000,'bin_pt'=>0.00000000000000000,'name'=>'sm_PktTemplate0_addr','width'=>6.00000000000000000},{'arith_type'=>2,'bin_pt'=>0,'name'=>'sm_PktTemplate0_din','width'=>32},{'arith_type'=>2.00000000000000000,'bin_pt'=>0.00000000000000000,'name'=>'sm_PktTemplate0_we','width'=>0.00000000000000000},{'arith_type'=>1.00000000000000000,'bin_pt'=>0.00000000000000000,'name'=>'shram_en','width'=>0.00000000000000000}]}  inheritDeviceType=inheritDeviceType  block_type=edkcore
      | library IEEE;
      | use IEEE.std_logic_1164.all;
      | use IEEE.numeric_std.all;
      | 
      | entity axi_sgiface is
      |     generic (
      |         -- AXI specific.
      |         -- TODO: need to figure out a way to pass these generics from outside
      |         C_S_AXI_SUPPORT_BURST   : integer := 0;
      |         -- TODO: fix the internal ID width to 8
      |         C_S_AXI_ID_WIDTH        : integer := 8;
      |         C_S_AXI_DATA_WIDTH      : integer := 32;
      |         C_S_AXI_ADDR_WIDTH      : integer := 32;
      |         C_S_AXI_TOTAL_ADDR_LEN  : integer := 12;
      |         C_S_AXI_LINEAR_ADDR_LEN : integer := 8;
      |         C_S_AXI_BANK_ADDR_LEN   : integer := 2;
      |         C_S_AXI_AWLEN_WIDTH     : integer := 8;
      |         C_S_AXI_ARLEN_WIDTH     : integer := 8
      |     );
      |     port (
      |         -- General.
      |         AXI_AClk      : in  std_logic;
      |         AXI_AResetN    : in  std_logic;
      |         -- not used
      |         AXI_Ce        : in  std_logic;
      |   
      |         -- AXI Port.
      |         S_AXI_AWADDR  : in  std_logic_vector(C_S_AXI_ADDR_WIDTH-1 downto 0);
      |         S_AXI_AWID    : in  std_logic_vector(C_S_AXI_ID_WIDTH-1 downto 0);
      |         S_AXI_AWLEN   : in  std_logic_vector(C_S_AXI_AWLEN_WIDTH-1 downto 0);
      |         S_AXI_AWSIZE  : in  std_logic_vector(2 downto 0);
      |         S_AXI_AWBURST : in  std_logic_vector(1 downto 0);
      |         S_AXI_AWLOCK  : in  std_logic_vector(1 downto 0);
      |         S_AXI_AWCACHE : in  std_logic_vector(3 downto 0);
      |         S_AXI_AWPROT  : in  std_logic_vector(2 downto 0);
      |         S_AXI_AWVALID : in  std_logic;
      |         S_AXI_AWREADY : out std_logic;
      |         
      |         S_AXI_WLAST   : in  std_logic;
      |         S_AXI_WDATA   : in  std_logic_vector(C_S_AXI_DATA_WIDTH-1 downto 0);
      |         S_AXI_WSTRB   : in  std_logic_vector((C_S_AXI_DATA_WIDTH/8)-1 downto 0);
      |         S_AXI_WVALID  : in  std_logic;
      |         S_AXI_WREADY  : out std_logic;
      |         
      |         S_AXI_BRESP   : out std_logic_vector(1 downto 0);
      |         S_AXI_BID     : out std_logic_vector(C_S_AXI_ID_WIDTH-1 downto 0);
      |         S_AXI_BVALID  : out std_logic;
      |         S_AXI_BREADY  : in  std_logic;
      |         
      |         S_AXI_ARADDR  : in  std_logic_vector(C_S_AXI_ADDR_WIDTH-1 downto 0);
      |         S_AXI_ARID    : in  std_logic_vector(C_S_AXI_ID_WIDTH-1 downto 0);
      |         S_AXI_ARLEN   : in  std_logic_vector(C_S_AXI_ARLEN_WIDTH-1 downto 0);
      |         S_AXI_ARSIZE  : in  std_logic_vector(2 downto 0);
      |         S_AXI_ARBURST : in  std_logic_vector(1 downto 0);
      |         S_AXI_ARLOCK  : in  std_logic_vector(1 downto 0);
      |         S_AXI_ARCACHE : in  std_logic_vector(3 downto 0);
      |         S_AXI_ARPROT  : in  std_logic_vector(2 downto 0);
      |         S_AXI_ARVALID : in  std_logic;
      |         S_AXI_ARREADY : out std_logic;
      |         
      |         -- 'From Register'
      |         -- 'CORE_INFO'
      |         sm_CORE_INFO_dout : in std_logic_vector(24-1 downto 0);
      |         -- 'TRIG_OUT'
      |         sm_TRIG_OUT_dout : in std_logic_vector(6-1 downto 0);
      |         -- 'To Register'
      |         -- 'TRIG_ODELAY_CFG_CMPLL'
      |         sm_TRIG_ODELAY_CFG_CMPLL_dout : in std_logic_vector(32-1 downto 0);
      |         sm_TRIG_ODELAY_CFG_CMPLL_din  : out std_logic_vector(32-1 downto 0);
      |         sm_TRIG_ODELAY_CFG_CMPLL_en   : out std_logic;
      |         -- 'TRIG_IDELAY_CFG_CMPLL'
      |         sm_TRIG_IDELAY_CFG_CMPLL_dout : in std_logic_vector(32-1 downto 0);
      |         sm_TRIG_IDELAY_CFG_CMPLL_din  : out std_logic_vector(32-1 downto 0);
      |         sm_TRIG_IDELAY_CFG_CMPLL_en   : out std_logic;
      |         -- 'TRIG_ODELAY_CFG_DEBUG_HDR'
      |         sm_TRIG_ODELAY_CFG_DEBUG_HDR_dout : in std_logic_vector(32-1 downto 0);
      |         sm_TRIG_ODELAY_CFG_DEBUG_HDR_din  : out std_logic_vector(32-1 downto 0);
      |         sm_TRIG_ODELAY_CFG_DEBUG_HDR_en   : out std_logic;
      |         -- 'TRIG_IDELAY_CFG_DEBUG_HDR'
      |         sm_TRIG_IDELAY_CFG_DEBUG_HDR_dout : in std_logic_vector(32-1 downto 0);
      |         sm_TRIG_IDELAY_CFG_DEBUG_HDR_din  : out std_logic_vector(32-1 downto 0);
      |         sm_TRIG_IDELAY_CFG_DEBUG_HDR_en   : out std_logic;
      |         -- 'TRIG_IODELAYS_CONTROL'
      |         sm_TRIG_IODELAYS_CONTROL_dout : in std_logic_vector(32-1 downto 0);
      |         sm_TRIG_IODELAYS_CONTROL_din  : out std_logic_vector(32-1 downto 0);
      |         sm_TRIG_IODELAYS_CONTROL_en   : out std_logic;
      |         -- 'RSSI_PKT_DET_CONFIG'
      |         sm_RSSI_PKT_DET_CONFIG_dout : in std_logic_vector(32-1 downto 0);
      |         sm_RSSI_PKT_DET_CONFIG_din  : out std_logic_vector(32-1 downto 0);
      |         sm_RSSI_PKT_DET_CONFIG_en   : out std_logic;
      |         -- 'TRIG_IN_CONF_6'
      |         sm_TRIG_IN_CONF_6_dout : in std_logic_vector(32-1 downto 0);
      |         sm_TRIG_IN_CONF_6_din  : out std_logic_vector(32-1 downto 0);
      |         sm_TRIG_IN_CONF_6_en   : out std_logic;
      |         -- 'TRIG_IN_CONF_5'
      |         sm_TRIG_IN_CONF_5_dout : in std_logic_vector(32-1 downto 0);
      |         sm_TRIG_IN_CONF_5_din  : out std_logic_vector(32-1 downto 0);
      |         sm_TRIG_IN_CONF_5_en   : out std_logic;
      |         -- 'TRIG_IN_CONF_4'
      |         sm_TRIG_IN_CONF_4_dout : in std_logic_vector(32-1 downto 0);
      |         sm_TRIG_IN_CONF_4_din  : out std_logic_vector(32-1 downto 0);
      |         sm_TRIG_IN_CONF_4_en   : out std_logic;
      |         -- 'TRIG_IN_CONF_3'
      |         sm_TRIG_IN_CONF_3_dout : in std_logic_vector(32-1 downto 0);
      |         sm_TRIG_IN_CONF_3_din  : out std_logic_vector(32-1 downto 0);
      |         sm_TRIG_IN_CONF_3_en   : out std_logic;
      |         -- 'TRIG_IN_CONF_2'
      |         sm_TRIG_IN_CONF_2_dout : in std_logic_vector(32-1 downto 0);
      |         sm_TRIG_IN_CONF_2_din  : out std_logic_vector(32-1 downto 0);
      |         sm_TRIG_IN_CONF_2_en   : out std_logic;
      |         -- 'TRIG_IN_CONF_0'
      |         sm_TRIG_IN_CONF_0_dout : in std_logic_vector(32-1 downto 0);
      |         sm_TRIG_IN_CONF_0_din  : out std_logic_vector(32-1 downto 0);
      |         sm_TRIG_IN_CONF_0_en   : out std_logic;
      |         -- 'TRIG_IN_CONF_8'
      |         sm_TRIG_IN_CONF_8_dout : in std_logic_vector(32-1 downto 0);
      |         sm_TRIG_IN_CONF_8_din  : out std_logic_vector(32-1 downto 0);
      |         sm_TRIG_IN_CONF_8_en   : out std_logic;
      |         -- 'TRIG_IN_CONF_7'
      |         sm_TRIG_IN_CONF_7_dout : in std_logic_vector(32-1 downto 0);
      |         sm_TRIG_IN_CONF_7_din  : out std_logic_vector(32-1 downto 0);
      |         sm_TRIG_IN_CONF_7_en   : out std_logic;
      |         -- 'TRIG_OUT_5_CONF_0'
      |         sm_TRIG_OUT_5_CONF_0_dout : in std_logic_vector(32-1 downto 0);
      |         sm_TRIG_OUT_5_CONF_0_din  : out std_logic_vector(32-1 downto 0);
      |         sm_TRIG_OUT_5_CONF_0_en   : out std_logic;
      |         -- 'TRIG_OUT_5_CONF_1'
      |         sm_TRIG_OUT_5_CONF_1_dout : in std_logic_vector(32-1 downto 0);
      |         sm_TRIG_OUT_5_CONF_1_din  : out std_logic_vector(32-1 downto 0);
      |         sm_TRIG_OUT_5_CONF_1_en   : out std_logic;
      |         -- 'TRIG_OUT_4_CONF_0'
      |         sm_TRIG_OUT_4_CONF_0_dout : in std_logic_vector(32-1 downto 0);
      |         sm_TRIG_OUT_4_CONF_0_din  : out std_logic_vector(32-1 downto 0);
      |         sm_TRIG_OUT_4_CONF_0_en   : out std_logic;
      |         -- 'TRIG_OUT_0_CONF_0'
      |         sm_TRIG_OUT_0_CONF_0_dout : in std_logic_vector(32-1 downto 0);
      |         sm_TRIG_OUT_0_CONF_0_din  : out std_logic_vector(32-1 downto 0);
      |         sm_TRIG_OUT_0_CONF_0_en   : out std_logic;
      |         -- 'TRIG_OUT_4_CONF_1'
      |         sm_TRIG_OUT_4_CONF_1_dout : in std_logic_vector(32-1 downto 0);
      |         sm_TRIG_OUT_4_CONF_1_din  : out std_logic_vector(32-1 downto 0);
      |         sm_TRIG_OUT_4_CONF_1_en   : out std_logic;
      |         -- 'TRIG_OUT_3_CONF_0'
      |         sm_TRIG_OUT_3_CONF_0_dout : in std_logic_vector(32-1 downto 0);
      |         sm_TRIG_OUT_3_CONF_0_din  : out std_logic_vector(32-1 downto 0);
      |         sm_TRIG_OUT_3_CONF_0_en   : out std_logic;
      |         -- 'TRIG_OUT_3_CONF_1'
      |         sm_TRIG_OUT_3_CONF_1_dout : in std_logic_vector(32-1 downto 0);
      |         sm_TRIG_OUT_3_CONF_1_din  : out std_logic_vector(32-1 downto 0);
      |         sm_TRIG_OUT_3_CONF_1_en   : out std_logic;
      |         -- 'TRIG_OUT_2_CONF_0'
      |         sm_TRIG_OUT_2_CONF_0_dout : in std_logic_vector(32-1 downto 0);
      |         sm_TRIG_OUT_2_CONF_0_din  : out std_logic_vector(32-1 downto 0);
      |         sm_TRIG_OUT_2_CONF_0_en   : out std_logic;
      |         -- 'TRIG_OUT_2_CONF_1'
      |         sm_TRIG_OUT_2_CONF_1_dout : in std_logic_vector(32-1 downto 0);
      |         sm_TRIG_OUT_2_CONF_1_din  : out std_logic_vector(32-1 downto 0);
      |         sm_TRIG_OUT_2_CONF_1_en   : out std_logic;
      |         -- 'TRIG_OUT_1_CONF_0'
      |         sm_TRIG_OUT_1_CONF_0_dout : in std_logic_vector(32-1 downto 0);
      |         sm_TRIG_OUT_1_CONF_0_din  : out std_logic_vector(32-1 downto 0);
      |         sm_TRIG_OUT_1_CONF_0_en   : out std_logic;
      |         -- 'TRIG_OUT_1_CONF_1'
      |         sm_TRIG_OUT_1_CONF_1_dout : in std_logic_vector(32-1 downto 0);
      |         sm_TRIG_OUT_1_CONF_1_din  : out std_logic_vector(32-1 downto 0);
      |         sm_TRIG_OUT_1_CONF_1_en   : out std_logic;
      |         -- 'TRIG_OUT_0_CONF_1'
      |         sm_TRIG_OUT_0_CONF_1_dout : in std_logic_vector(32-1 downto 0);
      |         sm_TRIG_OUT_0_CONF_1_din  : out std_logic_vector(32-1 downto 0);
      |         sm_TRIG_OUT_0_CONF_1_en   : out std_logic;
      |         -- 'RSSI_PKT_DET_DURATIONS'
      |         sm_RSSI_PKT_DET_DURATIONS_dout : in std_logic_vector(32-1 downto 0);
      |         sm_RSSI_PKT_DET_DURATIONS_din  : out std_logic_vector(32-1 downto 0);
      |         sm_RSSI_PKT_DET_DURATIONS_en   : out std_logic;
      |         -- 'RSSI_PKT_DET_THRESHOLDS'
      |         sm_RSSI_PKT_DET_THRESHOLDS_dout : in std_logic_vector(32-1 downto 0);
      |         sm_RSSI_PKT_DET_THRESHOLDS_din  : out std_logic_vector(32-1 downto 0);
      |         sm_RSSI_PKT_DET_THRESHOLDS_en   : out std_logic;
      |         -- 'TRIG_IN_CONF_1'
      |         sm_TRIG_IN_CONF_1_dout : in std_logic_vector(32-1 downto 0);
      |         sm_TRIG_IN_CONF_1_din  : out std_logic_vector(32-1 downto 0);
      |         sm_TRIG_IN_CONF_1_en   : out std_logic;
      |         -- 'From FIFO'
      |         -- 'To FIFO'
      |         -- 'Shared Memory'
      |         -- 'PktOps1'
      |         sm_PktOps1_dout  : in  std_logic_vector(32-1 downto 0);
      |         sm_PktOps1_addr  : out std_logic_vector(6-1 downto 0);
      |         sm_PktOps1_din   : out std_logic_vector(32-1 downto 0);
      |         sm_PktOps1_we    : out std_logic;
      |         -- 'PktTemplate1'
      |         sm_PktTemplate1_dout  : in  std_logic_vector(32-1 downto 0);
      |         sm_PktTemplate1_addr  : out std_logic_vector(6-1 downto 0);
      |         sm_PktTemplate1_din   : out std_logic_vector(32-1 downto 0);
      |         sm_PktTemplate1_we    : out std_logic;
      |         -- 'PktOps0'
      |         sm_PktOps0_dout  : in  std_logic_vector(32-1 downto 0);
      |         sm_PktOps0_addr  : out std_logic_vector(6-1 downto 0);
      |         sm_PktOps0_din   : out std_logic_vector(32-1 downto 0);
      |         sm_PktOps0_we    : out std_logic;
      |         -- 'PktTemplate0'
      |         sm_PktTemplate0_dout  : in  std_logic_vector(32-1 downto 0);
      |         sm_PktTemplate0_addr  : out std_logic_vector(6-1 downto 0);
      |         sm_PktTemplate0_din   : out std_logic_vector(32-1 downto 0);
      |         sm_PktTemplate0_we    : out std_logic;
      |         shram_en : out std_logic;
      | 
      |         S_AXI_RLAST   : out std_logic;
      |         S_AXI_RID     : out std_logic_vector(C_S_AXI_ID_WIDTH-1 downto 0);
      |         S_AXI_RDATA   : out std_logic_vector(C_S_AXI_DATA_WIDTH-1 downto 0);
      |         S_AXI_RRESP   : out std_logic_vector(1 downto 0);
      |         S_AXI_RVALID  : out std_logic;
      |         S_AXI_RREADY  : in  std_logic
      |     );
      | end entity axi_sgiface;
      | 
      | architecture IMP of axi_sgiface is
      | 
      | -- Internal signals for write channel.
      | signal S_AXI_BVALID_i       : std_logic;
      | signal S_AXI_BID_i          : std_logic_vector(C_S_AXI_ID_WIDTH-1 downto 0);
      | signal S_AXI_WREADY_i       : std_logic;
      |   
      | -- Internal signals for read channels.
      | signal S_AXI_ARLEN_i        : std_logic_vector(C_S_AXI_ARLEN_WIDTH-1 downto 0);
      | signal S_AXI_RLAST_i        : std_logic;
      | signal S_AXI_RREADY_i       : std_logic;
      | signal S_AXI_RVALID_i       : std_logic;
      | signal S_AXI_RDATA_i        : std_logic_vector(C_S_AXI_DATA_WIDTH-1 downto 0);
      | signal S_AXI_RID_i          : std_logic_vector(C_S_AXI_ID_WIDTH-1 downto 0);
      | 
      | -- for read channel
      | signal read_bank_addr_i     : std_logic_vector(C_S_AXI_BANK_ADDR_LEN-1 downto 0);
      | signal read_linear_addr_i   : std_logic_vector(C_S_AXI_LINEAR_ADDR_LEN-1 downto 0);
      | -- for write channel
      | signal write_bank_addr_i    : std_logic_vector(C_S_AXI_BANK_ADDR_LEN-1 downto 0);
      | signal write_linear_addr_i  : std_logic_vector(C_S_AXI_LINEAR_ADDR_LEN-1 downto 0);
      | 
      | signal reg_bank_out_i       : std_logic_vector(C_S_AXI_DATA_WIDTH-1 downto 0);
      | signal fifo_bank_out_i      : std_logic_vector(C_S_AXI_DATA_WIDTH-1 downto 0);
      | signal shmem_bank_out_i     : std_logic_vector(C_S_AXI_DATA_WIDTH-1 downto 0);
      |     
      | -- 'From Register'
      | -- 'CORE_INFO'
      | signal sm_CORE_INFO_dout_i  : std_logic_vector(C_S_AXI_DATA_WIDTH-1 downto 0);
      | -- 'TRIG_OUT'
      | signal sm_TRIG_OUT_dout_i  : std_logic_vector(C_S_AXI_DATA_WIDTH-1 downto 0);
      | -- 'To Register'
      | -- 'TRIG_ODELAY_CFG_CMPLL'
      | signal sm_TRIG_ODELAY_CFG_CMPLL_din_i   : std_logic_vector(C_S_AXI_DATA_WIDTH-1 downto 0);
      | signal sm_TRIG_ODELAY_CFG_CMPLL_en_i    : std_logic;
      | signal sm_TRIG_ODELAY_CFG_CMPLL_dout_i  : std_logic_vector(C_S_AXI_DATA_WIDTH-1 downto 0);
      | -- 'TRIG_IDELAY_CFG_CMPLL'
      | signal sm_TRIG_IDELAY_CFG_CMPLL_din_i   : std_logic_vector(C_S_AXI_DATA_WIDTH-1 downto 0);
      | signal sm_TRIG_IDELAY_CFG_CMPLL_en_i    : std_logic;
      | signal sm_TRIG_IDELAY_CFG_CMPLL_dout_i  : std_logic_vector(C_S_AXI_DATA_WIDTH-1 downto 0);
      | -- 'TRIG_ODELAY_CFG_DEBUG_HDR'
      | signal sm_TRIG_ODELAY_CFG_DEBUG_HDR_din_i   : std_logic_vector(C_S_AXI_DATA_WIDTH-1 downto 0);
      | signal sm_TRIG_ODELAY_CFG_DEBUG_HDR_en_i    : std_logic;
      | signal sm_TRIG_ODELAY_CFG_DEBUG_HDR_dout_i  : std_logic_vector(C_S_AXI_DATA_WIDTH-1 downto 0);
      | -- 'TRIG_IDELAY_CFG_DEBUG_HDR'
      | signal sm_TRIG_IDELAY_CFG_DEBUG_HDR_din_i   : std_logic_vector(C_S_AXI_DATA_WIDTH-1 downto 0);
      | signal sm_TRIG_IDELAY_CFG_DEBUG_HDR_en_i    : std_logic;
      | signal sm_TRIG_IDELAY_CFG_DEBUG_HDR_dout_i  : std_logic_vector(C_S_AXI_DATA_WIDTH-1 downto 0);
      | -- 'TRIG_IODELAYS_CONTROL'
      | signal sm_TRIG_IODELAYS_CONTROL_din_i   : std_logic_vector(C_S_AXI_DATA_WIDTH-1 downto 0);
      | signal sm_TRIG_IODELAYS_CONTROL_en_i    : std_logic;
      | signal sm_TRIG_IODELAYS_CONTROL_dout_i  : std_logic_vector(C_S_AXI_DATA_WIDTH-1 downto 0);
      | -- 'RSSI_PKT_DET_CONFIG'
      | signal sm_RSSI_PKT_DET_CONFIG_din_i   : std_logic_vector(C_S_AXI_DATA_WIDTH-1 downto 0);
      | signal sm_RSSI_PKT_DET_CONFIG_en_i    : std_logic;
      | signal sm_RSSI_PKT_DET_CONFIG_dout_i  : std_logic_vector(C_S_AXI_DATA_WIDTH-1 downto 0);
      | -- 'TRIG_IN_CONF_6'
      | signal sm_TRIG_IN_CONF_6_din_i   : std_logic_vector(C_S_AXI_DATA_WIDTH-1 downto 0);
      | signal sm_TRIG_IN_CONF_6_en_i    : std_logic;
      | signal sm_TRIG_IN_CONF_6_dout_i  : std_logic_vector(C_S_AXI_DATA_WIDTH-1 downto 0);
      | -- 'TRIG_IN_CONF_5'
      | signal sm_TRIG_IN_CONF_5_din_i   : std_logic_vector(C_S_AXI_DATA_WIDTH-1 downto 0);
      | signal sm_TRIG_IN_CONF_5_en_i    : std_logic;
      | signal sm_TRIG_IN_CONF_5_dout_i  : std_logic_vector(C_S_AXI_DATA_WIDTH-1 downto 0);
      | -- 'TRIG_IN_CONF_4'
      | signal sm_TRIG_IN_CONF_4_din_i   : std_logic_vector(C_S_AXI_DATA_WIDTH-1 downto 0);
      | signal sm_TRIG_IN_CONF_4_en_i    : std_logic;
      | signal sm_TRIG_IN_CONF_4_dout_i  : std_logic_vector(C_S_AXI_DATA_WIDTH-1 downto 0);
      | -- 'TRIG_IN_CONF_3'
      | signal sm_TRIG_IN_CONF_3_din_i   : std_logic_vector(C_S_AXI_DATA_WIDTH-1 downto 0);
      | signal sm_TRIG_IN_CONF_3_en_i    : std_logic;
      | signal sm_TRIG_IN_CONF_3_dout_i  : std_logic_vector(C_S_AXI_DATA_WIDTH-1 downto 0);
      | -- 'TRIG_IN_CONF_2'
      | signal sm_TRIG_IN_CONF_2_din_i   : std_logic_vector(C_S_AXI_DATA_WIDTH-1 downto 0);
      | signal sm_TRIG_IN_CONF_2_en_i    : std_logic;
      | signal sm_TRIG_IN_CONF_2_dout_i  : std_logic_vector(C_S_AXI_DATA_WIDTH-1 downto 0);
      | -- 'TRIG_IN_CONF_0'
      | signal sm_TRIG_IN_CONF_0_din_i   : std_logic_vector(C_S_AXI_DATA_WIDTH-1 downto 0);
      | signal sm_TRIG_IN_CONF_0_en_i    : std_logic;
      | signal sm_TRIG_IN_CONF_0_dout_i  : std_logic_vector(C_S_AXI_DATA_WIDTH-1 downto 0);
      | -- 'TRIG_IN_CONF_8'
      | signal sm_TRIG_IN_CONF_8_din_i   : std_logic_vector(C_S_AXI_DATA_WIDTH-1 downto 0);
      | signal sm_TRIG_IN_CONF_8_en_i    : std_logic;
      | signal sm_TRIG_IN_CONF_8_dout_i  : std_logic_vector(C_S_AXI_DATA_WIDTH-1 downto 0);
      | -- 'TRIG_IN_CONF_7'
      | signal sm_TRIG_IN_CONF_7_din_i   : std_logic_vector(C_S_AXI_DATA_WIDTH-1 downto 0);
      | signal sm_TRIG_IN_CONF_7_en_i    : std_logic;
      | signal sm_TRIG_IN_CONF_7_dout_i  : std_logic_vector(C_S_AXI_DATA_WIDTH-1 downto 0);
      | -- 'TRIG_OUT_5_CONF_0'
      | signal sm_TRIG_OUT_5_CONF_0_din_i   : std_logic_vector(C_S_AXI_DATA_WIDTH-1 downto 0);
      | signal sm_TRIG_OUT_5_CONF_0_en_i    : std_logic;
      | signal sm_TRIG_OUT_5_CONF_0_dout_i  : std_logic_vector(C_S_AXI_DATA_WIDTH-1 downto 0);
      | -- 'TRIG_OUT_5_CONF_1'
      | signal sm_TRIG_OUT_5_CONF_1_din_i   : std_logic_vector(C_S_AXI_DATA_WIDTH-1 downto 0);
      | signal sm_TRIG_OUT_5_CONF_1_en_i    : std_logic;
      | signal sm_TRIG_OUT_5_CONF_1_dout_i  : std_logic_vector(C_S_AXI_DATA_WIDTH-1 downto 0);
      | -- 'TRIG_OUT_4_CONF_0'
      | signal sm_TRIG_OUT_4_CONF_0_din_i   : std_logic_vector(C_S_AXI_DATA_WIDTH-1 downto 0);
      | signal sm_TRIG_OUT_4_CONF_0_en_i    : std_logic;
      | signal sm_TRIG_OUT_4_CONF_0_dout_i  : std_logic_vector(C_S_AXI_DATA_WIDTH-1 downto 0);
      | -- 'TRIG_OUT_0_CONF_0'
      | signal sm_TRIG_OUT_0_CONF_0_din_i   : std_logic_vector(C_S_AXI_DATA_WIDTH-1 downto 0);
      | signal sm_TRIG_OUT_0_CONF_0_en_i    : std_logic;
      | signal sm_TRIG_OUT_0_CONF_0_dout_i  : std_logic_vector(C_S_AXI_DATA_WIDTH-1 downto 0);
      | -- 'TRIG_OUT_4_CONF_1'
      | signal sm_TRIG_OUT_4_CONF_1_din_i   : std_logic_vector(C_S_AXI_DATA_WIDTH-1 downto 0);
      | signal sm_TRIG_OUT_4_CONF_1_en_i    : std_logic;
      | signal sm_TRIG_OUT_4_CONF_1_dout_i  : std_logic_vector(C_S_AXI_DATA_WIDTH-1 downto 0);
      | -- 'TRIG_OUT_3_CONF_0'
      | signal sm_TRIG_OUT_3_CONF_0_din_i   : std_logic_vector(C_S_AXI_DATA_WIDTH-1 downto 0);
      | signal sm_TRIG_OUT_3_CONF_0_en_i    : std_logic;
      | signal sm_TRIG_OUT_3_CONF_0_dout_i  : std_logic_vector(C_S_AXI_DATA_WIDTH-1 downto 0);
      | -- 'TRIG_OUT_3_CONF_1'
      | signal sm_TRIG_OUT_3_CONF_1_din_i   : std_logic_vector(C_S_AXI_DATA_WIDTH-1 downto 0);
      | signal sm_TRIG_OUT_3_CONF_1_en_i    : std_logic;
      | signal sm_TRIG_OUT_3_CONF_1_dout_i  : std_logic_vector(C_S_AXI_DATA_WIDTH-1 downto 0);
      | -- 'TRIG_OUT_2_CONF_0'
      | signal sm_TRIG_OUT_2_CONF_0_din_i   : std_logic_vector(C_S_AXI_DATA_WIDTH-1 downto 0);
      | signal sm_TRIG_OUT_2_CONF_0_en_i    : std_logic;
      | signal sm_TRIG_OUT_2_CONF_0_dout_i  : std_logic_vector(C_S_AXI_DATA_WIDTH-1 downto 0);
      | -- 'TRIG_OUT_2_CONF_1'
      | signal sm_TRIG_OUT_2_CONF_1_din_i   : std_logic_vector(C_S_AXI_DATA_WIDTH-1 downto 0);
      | signal sm_TRIG_OUT_2_CONF_1_en_i    : std_logic;
      | signal sm_TRIG_OUT_2_CONF_1_dout_i  : std_logic_vector(C_S_AXI_DATA_WIDTH-1 downto 0);
      | -- 'TRIG_OUT_1_CONF_0'
      | signal sm_TRIG_OUT_1_CONF_0_din_i   : std_logic_vector(C_S_AXI_DATA_WIDTH-1 downto 0);
      | signal sm_TRIG_OUT_1_CONF_0_en_i    : std_logic;
      | signal sm_TRIG_OUT_1_CONF_0_dout_i  : std_logic_vector(C_S_AXI_DATA_WIDTH-1 downto 0);
      | -- 'TRIG_OUT_1_CONF_1'
      | signal sm_TRIG_OUT_1_CONF_1_din_i   : std_logic_vector(C_S_AXI_DATA_WIDTH-1 downto 0);
      | signal sm_TRIG_OUT_1_CONF_1_en_i    : std_logic;
      | signal sm_TRIG_OUT_1_CONF_1_dout_i  : std_logic_vector(C_S_AXI_DATA_WIDTH-1 downto 0);
      | -- 'TRIG_OUT_0_CONF_1'
      | signal sm_TRIG_OUT_0_CONF_1_din_i   : std_logic_vector(C_S_AXI_DATA_WIDTH-1 downto 0);
      | signal sm_TRIG_OUT_0_CONF_1_en_i    : std_logic;
      | signal sm_TRIG_OUT_0_CONF_1_dout_i  : std_logic_vector(C_S_AXI_DATA_WIDTH-1 downto 0);
      | -- 'RSSI_PKT_DET_DURATIONS'
      | signal sm_RSSI_PKT_DET_DURATIONS_din_i   : std_logic_vector(C_S_AXI_DATA_WIDTH-1 downto 0);
      | signal sm_RSSI_PKT_DET_DURATIONS_en_i    : std_logic;
      | signal sm_RSSI_PKT_DET_DURATIONS_dout_i  : std_logic_vector(C_S_AXI_DATA_WIDTH-1 downto 0);
      | -- 'RSSI_PKT_DET_THRESHOLDS'
      | signal sm_RSSI_PKT_DET_THRESHOLDS_din_i   : std_logic_vector(C_S_AXI_DATA_WIDTH-1 downto 0);
      | signal sm_RSSI_PKT_DET_THRESHOLDS_en_i    : std_logic;
      | signal sm_RSSI_PKT_DET_THRESHOLDS_dout_i  : std_logic_vector(C_S_AXI_DATA_WIDTH-1 downto 0);
      | -- 'TRIG_IN_CONF_1'
      | signal sm_TRIG_IN_CONF_1_din_i   : std_logic_vector(C_S_AXI_DATA_WIDTH-1 downto 0);
      | signal sm_TRIG_IN_CONF_1_en_i    : std_logic;
      | signal sm_TRIG_IN_CONF_1_dout_i  : std_logic_vector(C_S_AXI_DATA_WIDTH-1 downto 0);
      | -- 'From FIFO'
      | -- 'To FIFO'
      | -- 'Shared Memory'
      | -- 'PktOps1'
      | signal sm_PktOps1_addr_i  : std_logic_vector(C_S_AXI_LINEAR_ADDR_LEN-1 downto 0);
      | signal sm_PktOps1_din_i   : std_logic_vector(C_S_AXI_DATA_WIDTH-1 downto 0);
      | signal sm_PktOps1_we_i    : std_logic;
      | signal sm_PktOps1_dout_i  : std_logic_vector(C_S_AXI_DATA_WIDTH-1 downto 0);
      | -- 'PktTemplate1'
      | signal sm_PktTemplate1_addr_i  : std_logic_vector(C_S_AXI_LINEAR_ADDR_LEN-1 downto 0);
      | signal sm_PktTemplate1_din_i   : std_logic_vector(C_S_AXI_DATA_WIDTH-1 downto 0);
      | signal sm_PktTemplate1_we_i    : std_logic;
      | signal sm_PktTemplate1_dout_i  : std_logic_vector(C_S_AXI_DATA_WIDTH-1 downto 0);
      | -- 'PktOps0'
      | signal sm_PktOps0_addr_i  : std_logic_vector(C_S_AXI_LINEAR_ADDR_LEN-1 downto 0);
      | signal sm_PktOps0_din_i   : std_logic_vector(C_S_AXI_DATA_WIDTH-1 downto 0);
      | signal sm_PktOps0_we_i    : std_logic;
      | signal sm_PktOps0_dout_i  : std_logic_vector(C_S_AXI_DATA_WIDTH-1 downto 0);
      | -- 'PktTemplate0'
      | signal sm_PktTemplate0_addr_i  : std_logic_vector(C_S_AXI_LINEAR_ADDR_LEN-1 downto 0);
      | signal sm_PktTemplate0_din_i   : std_logic_vector(C_S_AXI_DATA_WIDTH-1 downto 0);
      | signal sm_PktTemplate0_we_i    : std_logic;
      | signal sm_PktTemplate0_dout_i  : std_logic_vector(C_S_AXI_DATA_WIDTH-1 downto 0);
      | 
      | type t_read_state is (IDLE, READ_PREP, READ_DATA);
      | signal read_state : t_read_state;
      | 
      | type t_write_state is (IDLE, WRITE_DATA, WRITE_RESPONSE);
      | signal write_state : t_write_state;
      | 
      | type t_memmap_state is (READ, WRITE);
      | signal memmap_state : t_memmap_state;
      | 
      | constant C_READ_PREP_DELAY : std_logic_vector(1 downto 0) := "11";
      | 
      | signal read_prep_counter : std_logic_vector(1 downto 0);
      | signal read_addr_counter : std_logic_vector(C_S_AXI_ARLEN_WIDTH-1 downto 0);
      | signal read_data_counter : std_logic_vector(C_S_AXI_ARLEN_WIDTH-1 downto 0);
      | 
      | -- enable of shared BRAMs
      | signal s_shram_en : std_logic;
      | 
      | signal write_addr_valid : std_logic;
      | signal write_ready : std_logic;
      | 
      | -- 're' of From/To FIFOs
      | signal s_fifo_re : std_logic;
      | -- 'we' of To FIFOs
      | signal s_fifo_we : std_logic;
      | 
      | begin
      | 
      | -- enable for 'Shared Memory' blocks
      | shram_en <= s_shram_en;
      | -- PktOps1 din
      | sm_PktOps1_din_i <= S_AXI_WDATA;
      | -- PktTemplate1 din
      | sm_PktTemplate1_din_i <= S_AXI_WDATA;
      | -- PktOps0 din
      | sm_PktOps0_din_i <= S_AXI_WDATA;
      | -- PktTemplate0 din
      | sm_PktTemplate0_din_i <= S_AXI_WDATA;
      | 
      | -- conversion to match with the data bus width
      | -- 'From Register'
      | -- 'CORE_INFO'
      | gen_sm_CORE_INFO_dout_i: if (24 < C_S_AXI_DATA_WIDTH) generate
      |     sm_CORE_INFO_dout_i(C_S_AXI_DATA_WIDTH-1 downto 24) <= (others => '0');
      | end generate gen_sm_CORE_INFO_dout_i;
      | sm_CORE_INFO_dout_i(24-1 downto 0) <= sm_CORE_INFO_dout;
      | -- 'TRIG_OUT'
      | gen_sm_TRIG_OUT_dout_i: if (6 < C_S_AXI_DATA_WIDTH) generate
      |     sm_TRIG_OUT_dout_i(C_S_AXI_DATA_WIDTH-1 downto 6) <= (others => '0');
      | end generate gen_sm_TRIG_OUT_dout_i;
      | sm_TRIG_OUT_dout_i(6-1 downto 0) <= sm_TRIG_OUT_dout;
      | -- 'To Register'
      | -- 'TRIG_ODELAY_CFG_CMPLL'
      | sm_TRIG_ODELAY_CFG_CMPLL_din     <= sm_TRIG_ODELAY_CFG_CMPLL_din_i(32-1 downto 0);
      | sm_TRIG_ODELAY_CFG_CMPLL_en      <= sm_TRIG_ODELAY_CFG_CMPLL_en_i;
      | gen_sm_TRIG_ODELAY_CFG_CMPLL_dout_i: if (32 < C_S_AXI_DATA_WIDTH) generate
      |     sm_TRIG_ODELAY_CFG_CMPLL_dout_i(C_S_AXI_DATA_WIDTH-1 downto 32) <= (others => '0');
      | end generate gen_sm_TRIG_ODELAY_CFG_CMPLL_dout_i;
      | sm_TRIG_ODELAY_CFG_CMPLL_dout_i(32-1 downto 0) <= sm_TRIG_ODELAY_CFG_CMPLL_dout;
      | -- 'TRIG_IDELAY_CFG_CMPLL'
      | sm_TRIG_IDELAY_CFG_CMPLL_din     <= sm_TRIG_IDELAY_CFG_CMPLL_din_i(32-1 downto 0);
      | sm_TRIG_IDELAY_CFG_CMPLL_en      <= sm_TRIG_IDELAY_CFG_CMPLL_en_i;
      | gen_sm_TRIG_IDELAY_CFG_CMPLL_dout_i: if (32 < C_S_AXI_DATA_WIDTH) generate
      |     sm_TRIG_IDELAY_CFG_CMPLL_dout_i(C_S_AXI_DATA_WIDTH-1 downto 32) <= (others => '0');
      | end generate gen_sm_TRIG_IDELAY_CFG_CMPLL_dout_i;
      | sm_TRIG_IDELAY_CFG_CMPLL_dout_i(32-1 downto 0) <= sm_TRIG_IDELAY_CFG_CMPLL_dout;
      | -- 'TRIG_ODELAY_CFG_DEBUG_HDR'
      | sm_TRIG_ODELAY_CFG_DEBUG_HDR_din     <= sm_TRIG_ODELAY_CFG_DEBUG_HDR_din_i(32-1 downto 0);
      | sm_TRIG_ODELAY_CFG_DEBUG_HDR_en      <= sm_TRIG_ODELAY_CFG_DEBUG_HDR_en_i;
      | gen_sm_TRIG_ODELAY_CFG_DEBUG_HDR_dout_i: if (32 < C_S_AXI_DATA_WIDTH) generate
      |     sm_TRIG_ODELAY_CFG_DEBUG_HDR_dout_i(C_S_AXI_DATA_WIDTH-1 downto 32) <= (others => '0');
      | end generate gen_sm_TRIG_ODELAY_CFG_DEBUG_HDR_dout_i;
      | sm_TRIG_ODELAY_CFG_DEBUG_HDR_dout_i(32-1 downto 0) <= sm_TRIG_ODELAY_CFG_DEBUG_HDR_dout;
      | -- 'TRIG_IDELAY_CFG_DEBUG_HDR'
      | sm_TRIG_IDELAY_CFG_DEBUG_HDR_din     <= sm_TRIG_IDELAY_CFG_DEBUG_HDR_din_i(32-1 downto 0);
      | sm_TRIG_IDELAY_CFG_DEBUG_HDR_en      <= sm_TRIG_IDELAY_CFG_DEBUG_HDR_en_i;
      | gen_sm_TRIG_IDELAY_CFG_DEBUG_HDR_dout_i: if (32 < C_S_AXI_DATA_WIDTH) generate
      |     sm_TRIG_IDELAY_CFG_DEBUG_HDR_dout_i(C_S_AXI_DATA_WIDTH-1 downto 32) <= (others => '0');
      | end generate gen_sm_TRIG_IDELAY_CFG_DEBUG_HDR_dout_i;
      | sm_TRIG_IDELAY_CFG_DEBUG_HDR_dout_i(32-1 downto 0) <= sm_TRIG_IDELAY_CFG_DEBUG_HDR_dout;
      | -- 'TRIG_IODELAYS_CONTROL'
      | sm_TRIG_IODELAYS_CONTROL_din     <= sm_TRIG_IODELAYS_CONTROL_din_i(32-1 downto 0);
      | sm_TRIG_IODELAYS_CONTROL_en      <= sm_TRIG_IODELAYS_CONTROL_en_i;
      | gen_sm_TRIG_IODELAYS_CONTROL_dout_i: if (32 < C_S_AXI_DATA_WIDTH) generate
      |     sm_TRIG_IODELAYS_CONTROL_dout_i(C_S_AXI_DATA_WIDTH-1 downto 32) <= (others => '0');
      | end generate gen_sm_TRIG_IODELAYS_CONTROL_dout_i;
      | sm_TRIG_IODELAYS_CONTROL_dout_i(32-1 downto 0) <= sm_TRIG_IODELAYS_CONTROL_dout;
      | -- 'RSSI_PKT_DET_CONFIG'
      | sm_RSSI_PKT_DET_CONFIG_din     <= sm_RSSI_PKT_DET_CONFIG_din_i(32-1 downto 0);
      | sm_RSSI_PKT_DET_CONFIG_en      <= sm_RSSI_PKT_DET_CONFIG_en_i;
      | gen_sm_RSSI_PKT_DET_CONFIG_dout_i: if (32 < C_S_AXI_DATA_WIDTH) generate
      |     sm_RSSI_PKT_DET_CONFIG_dout_i(C_S_AXI_DATA_WIDTH-1 downto 32) <= (others => '0');
      | end generate gen_sm_RSSI_PKT_DET_CONFIG_dout_i;
      | sm_RSSI_PKT_DET_CONFIG_dout_i(32-1 downto 0) <= sm_RSSI_PKT_DET_CONFIG_dout;
      | -- 'TRIG_IN_CONF_6'
      | sm_TRIG_IN_CONF_6_din     <= sm_TRIG_IN_CONF_6_din_i(32-1 downto 0);
      | sm_TRIG_IN_CONF_6_en      <= sm_TRIG_IN_CONF_6_en_i;
      | gen_sm_TRIG_IN_CONF_6_dout_i: if (32 < C_S_AXI_DATA_WIDTH) generate
      |     sm_TRIG_IN_CONF_6_dout_i(C_S_AXI_DATA_WIDTH-1 downto 32) <= (others => '0');
      | end generate gen_sm_TRIG_IN_CONF_6_dout_i;
      | sm_TRIG_IN_CONF_6_dout_i(32-1 downto 0) <= sm_TRIG_IN_CONF_6_dout;
      | -- 'TRIG_IN_CONF_5'
      | sm_TRIG_IN_CONF_5_din     <= sm_TRIG_IN_CONF_5_din_i(32-1 downto 0);
      | sm_TRIG_IN_CONF_5_en      <= sm_TRIG_IN_CONF_5_en_i;
      | gen_sm_TRIG_IN_CONF_5_dout_i: if (32 < C_S_AXI_DATA_WIDTH) generate
      |     sm_TRIG_IN_CONF_5_dout_i(C_S_AXI_DATA_WIDTH-1 downto 32) <= (others => '0');
      | end generate gen_sm_TRIG_IN_CONF_5_dout_i;
      | sm_TRIG_IN_CONF_5_dout_i(32-1 downto 0) <= sm_TRIG_IN_CONF_5_dout;
      | -- 'TRIG_IN_CONF_4'
      | sm_TRIG_IN_CONF_4_din     <= sm_TRIG_IN_CONF_4_din_i(32-1 downto 0);
      | sm_TRIG_IN_CONF_4_en      <= sm_TRIG_IN_CONF_4_en_i;
      | gen_sm_TRIG_IN_CONF_4_dout_i: if (32 < C_S_AXI_DATA_WIDTH) generate
      |     sm_TRIG_IN_CONF_4_dout_i(C_S_AXI_DATA_WIDTH-1 downto 32) <= (others => '0');
      | end generate gen_sm_TRIG_IN_CONF_4_dout_i;
      | sm_TRIG_IN_CONF_4_dout_i(32-1 downto 0) <= sm_TRIG_IN_CONF_4_dout;
      | -- 'TRIG_IN_CONF_3'
      | sm_TRIG_IN_CONF_3_din     <= sm_TRIG_IN_CONF_3_din_i(32-1 downto 0);
      | sm_TRIG_IN_CONF_3_en      <= sm_TRIG_IN_CONF_3_en_i;
      | gen_sm_TRIG_IN_CONF_3_dout_i: if (32 < C_S_AXI_DATA_WIDTH) generate
      |     sm_TRIG_IN_CONF_3_dout_i(C_S_AXI_DATA_WIDTH-1 downto 32) <= (others => '0');
      | end generate gen_sm_TRIG_IN_CONF_3_dout_i;
      | sm_TRIG_IN_CONF_3_dout_i(32-1 downto 0) <= sm_TRIG_IN_CONF_3_dout;
      | -- 'TRIG_IN_CONF_2'
      | sm_TRIG_IN_CONF_2_din     <= sm_TRIG_IN_CONF_2_din_i(32-1 downto 0);
      | sm_TRIG_IN_CONF_2_en      <= sm_TRIG_IN_CONF_2_en_i;
      | gen_sm_TRIG_IN_CONF_2_dout_i: if (32 < C_S_AXI_DATA_WIDTH) generate
      |     sm_TRIG_IN_CONF_2_dout_i(C_S_AXI_DATA_WIDTH-1 downto 32) <= (others => '0');
      | end generate gen_sm_TRIG_IN_CONF_2_dout_i;
      | sm_TRIG_IN_CONF_2_dout_i(32-1 downto 0) <= sm_TRIG_IN_CONF_2_dout;
      | -- 'TRIG_IN_CONF_0'
      | sm_TRIG_IN_CONF_0_din     <= sm_TRIG_IN_CONF_0_din_i(32-1 downto 0);
      | sm_TRIG_IN_CONF_0_en      <= sm_TRIG_IN_CONF_0_en_i;
      | gen_sm_TRIG_IN_CONF_0_dout_i: if (32 < C_S_AXI_DATA_WIDTH) generate
      |     sm_TRIG_IN_CONF_0_dout_i(C_S_AXI_DATA_WIDTH-1 downto 32) <= (others => '0');
      | end generate gen_sm_TRIG_IN_CONF_0_dout_i;
      | sm_TRIG_IN_CONF_0_dout_i(32-1 downto 0) <= sm_TRIG_IN_CONF_0_dout;
      | -- 'TRIG_IN_CONF_8'
      | sm_TRIG_IN_CONF_8_din     <= sm_TRIG_IN_CONF_8_din_i(32-1 downto 0);
      | sm_TRIG_IN_CONF_8_en      <= sm_TRIG_IN_CONF_8_en_i;
      | gen_sm_TRIG_IN_CONF_8_dout_i: if (32 < C_S_AXI_DATA_WIDTH) generate
      |     sm_TRIG_IN_CONF_8_dout_i(C_S_AXI_DATA_WIDTH-1 downto 32) <= (others => '0');
      | end generate gen_sm_TRIG_IN_CONF_8_dout_i;
      | sm_TRIG_IN_CONF_8_dout_i(32-1 downto 0) <= sm_TRIG_IN_CONF_8_dout;
      | -- 'TRIG_IN_CONF_7'
      | sm_TRIG_IN_CONF_7_din     <= sm_TRIG_IN_CONF_7_din_i(32-1 downto 0);
      | sm_TRIG_IN_CONF_7_en      <= sm_TRIG_IN_CONF_7_en_i;
      | gen_sm_TRIG_IN_CONF_7_dout_i: if (32 < C_S_AXI_DATA_WIDTH) generate
      |     sm_TRIG_IN_CONF_7_dout_i(C_S_AXI_DATA_WIDTH-1 downto 32) <= (others => '0');
      | end generate gen_sm_TRIG_IN_CONF_7_dout_i;
      | sm_TRIG_IN_CONF_7_dout_i(32-1 downto 0) <= sm_TRIG_IN_CONF_7_dout;
      | -- 'TRIG_OUT_5_CONF_0'
      | sm_TRIG_OUT_5_CONF_0_din     <= sm_TRIG_OUT_5_CONF_0_din_i(32-1 downto 0);
      | sm_TRIG_OUT_5_CONF_0_en      <= sm_TRIG_OUT_5_CONF_0_en_i;
      | gen_sm_TRIG_OUT_5_CONF_0_dout_i: if (32 < C_S_AXI_DATA_WIDTH) generate
      |     sm_TRIG_OUT_5_CONF_0_dout_i(C_S_AXI_DATA_WIDTH-1 downto 32) <= (others => '0');
      | end generate gen_sm_TRIG_OUT_5_CONF_0_dout_i;
      | sm_TRIG_OUT_5_CONF_0_dout_i(32-1 downto 0) <= sm_TRIG_OUT_5_CONF_0_dout;
      | -- 'TRIG_OUT_5_CONF_1'
      | sm_TRIG_OUT_5_CONF_1_din     <= sm_TRIG_OUT_5_CONF_1_din_i(32-1 downto 0);
      | sm_TRIG_OUT_5_CONF_1_en      <= sm_TRIG_OUT_5_CONF_1_en_i;
      | gen_sm_TRIG_OUT_5_CONF_1_dout_i: if (32 < C_S_AXI_DATA_WIDTH) generate
      |     sm_TRIG_OUT_5_CONF_1_dout_i(C_S_AXI_DATA_WIDTH-1 downto 32) <= (others => '0');
      | end generate gen_sm_TRIG_OUT_5_CONF_1_dout_i;
      | sm_TRIG_OUT_5_CONF_1_dout_i(32-1 downto 0) <= sm_TRIG_OUT_5_CONF_1_dout;
      | -- 'TRIG_OUT_4_CONF_0'
      | sm_TRIG_OUT_4_CONF_0_din     <= sm_TRIG_OUT_4_CONF_0_din_i(32-1 downto 0);
      | sm_TRIG_OUT_4_CONF_0_en      <= sm_TRIG_OUT_4_CONF_0_en_i;
      | gen_sm_TRIG_OUT_4_CONF_0_dout_i: if (32 < C_S_AXI_DATA_WIDTH) generate
      |     sm_TRIG_OUT_4_CONF_0_dout_i(C_S_AXI_DATA_WIDTH-1 downto 32) <= (others => '0');
      | end generate gen_sm_TRIG_OUT_4_CONF_0_dout_i;
      | sm_TRIG_OUT_4_CONF_0_dout_i(32-1 downto 0) <= sm_TRIG_OUT_4_CONF_0_dout;
      | -- 'TRIG_OUT_0_CONF_0'
      | sm_TRIG_OUT_0_CONF_0_din     <= sm_TRIG_OUT_0_CONF_0_din_i(32-1 downto 0);
      | sm_TRIG_OUT_0_CONF_0_en      <= sm_TRIG_OUT_0_CONF_0_en_i;
      | gen_sm_TRIG_OUT_0_CONF_0_dout_i: if (32 < C_S_AXI_DATA_WIDTH) generate
      |     sm_TRIG_OUT_0_CONF_0_dout_i(C_S_AXI_DATA_WIDTH-1 downto 32) <= (others => '0');
      | end generate gen_sm_TRIG_OUT_0_CONF_0_dout_i;
      | sm_TRIG_OUT_0_CONF_0_dout_i(32-1 downto 0) <= sm_TRIG_OUT_0_CONF_0_dout;
      | -- 'TRIG_OUT_4_CONF_1'
      | sm_TRIG_OUT_4_CONF_1_din     <= sm_TRIG_OUT_4_CONF_1_din_i(32-1 downto 0);
      | sm_TRIG_OUT_4_CONF_1_en      <= sm_TRIG_OUT_4_CONF_1_en_i;
      | gen_sm_TRIG_OUT_4_CONF_1_dout_i: if (32 < C_S_AXI_DATA_WIDTH) generate
      |     sm_TRIG_OUT_4_CONF_1_dout_i(C_S_AXI_DATA_WIDTH-1 downto 32) <= (others => '0');
      | end generate gen_sm_TRIG_OUT_4_CONF_1_dout_i;
      | sm_TRIG_OUT_4_CONF_1_dout_i(32-1 downto 0) <= sm_TRIG_OUT_4_CONF_1_dout;
      | -- 'TRIG_OUT_3_CONF_0'
      | sm_TRIG_OUT_3_CONF_0_din     <= sm_TRIG_OUT_3_CONF_0_din_i(32-1 downto 0);
      | sm_TRIG_OUT_3_CONF_0_en      <= sm_TRIG_OUT_3_CONF_0_en_i;
      | gen_sm_TRIG_OUT_3_CONF_0_dout_i: if (32 < C_S_AXI_DATA_WIDTH) generate
      |     sm_TRIG_OUT_3_CONF_0_dout_i(C_S_AXI_DATA_WIDTH-1 downto 32) <= (others => '0');
      | end generate gen_sm_TRIG_OUT_3_CONF_0_dout_i;
      | sm_TRIG_OUT_3_CONF_0_dout_i(32-1 downto 0) <= sm_TRIG_OUT_3_CONF_0_dout;
      | -- 'TRIG_OUT_3_CONF_1'
      | sm_TRIG_OUT_3_CONF_1_din     <= sm_TRIG_OUT_3_CONF_1_din_i(32-1 downto 0);
      | sm_TRIG_OUT_3_CONF_1_en      <= sm_TRIG_OUT_3_CONF_1_en_i;
      | gen_sm_TRIG_OUT_3_CONF_1_dout_i: if (32 < C_S_AXI_DATA_WIDTH) generate
      |     sm_TRIG_OUT_3_CONF_1_dout_i(C_S_AXI_DATA_WIDTH-1 downto 32) <= (others => '0');
      | end generate gen_sm_TRIG_OUT_3_CONF_1_dout_i;
      | sm_TRIG_OUT_3_CONF_1_dout_i(32-1 downto 0) <= sm_TRIG_OUT_3_CONF_1_dout;
      | -- 'TRIG_OUT_2_CONF_0'
      | sm_TRIG_OUT_2_CONF_0_din     <= sm_TRIG_OUT_2_CONF_0_din_i(32-1 downto 0);
      | sm_TRIG_OUT_2_CONF_0_en      <= sm_TRIG_OUT_2_CONF_0_en_i;
      | gen_sm_TRIG_OUT_2_CONF_0_dout_i: if (32 < C_S_AXI_DATA_WIDTH) generate
      |     sm_TRIG_OUT_2_CONF_0_dout_i(C_S_AXI_DATA_WIDTH-1 downto 32) <= (others => '0');
      | end generate gen_sm_TRIG_OUT_2_CONF_0_dout_i;
      | sm_TRIG_OUT_2_CONF_0_dout_i(32-1 downto 0) <= sm_TRIG_OUT_2_CONF_0_dout;
      | -- 'TRIG_OUT_2_CONF_1'
      | sm_TRIG_OUT_2_CONF_1_din     <= sm_TRIG_OUT_2_CONF_1_din_i(32-1 downto 0);
      | sm_TRIG_OUT_2_CONF_1_en      <= sm_TRIG_OUT_2_CONF_1_en_i;
      | gen_sm_TRIG_OUT_2_CONF_1_dout_i: if (32 < C_S_AXI_DATA_WIDTH) generate
      |     sm_TRIG_OUT_2_CONF_1_dout_i(C_S_AXI_DATA_WIDTH-1 downto 32) <= (others => '0');
      | end generate gen_sm_TRIG_OUT_2_CONF_1_dout_i;
      | sm_TRIG_OUT_2_CONF_1_dout_i(32-1 downto 0) <= sm_TRIG_OUT_2_CONF_1_dout;
      | -- 'TRIG_OUT_1_CONF_0'
      | sm_TRIG_OUT_1_CONF_0_din     <= sm_TRIG_OUT_1_CONF_0_din_i(32-1 downto 0);
      | sm_TRIG_OUT_1_CONF_0_en      <= sm_TRIG_OUT_1_CONF_0_en_i;
      | gen_sm_TRIG_OUT_1_CONF_0_dout_i: if (32 < C_S_AXI_DATA_WIDTH) generate
      |     sm_TRIG_OUT_1_CONF_0_dout_i(C_S_AXI_DATA_WIDTH-1 downto 32) <= (others => '0');
      | end generate gen_sm_TRIG_OUT_1_CONF_0_dout_i;
      | sm_TRIG_OUT_1_CONF_0_dout_i(32-1 downto 0) <= sm_TRIG_OUT_1_CONF_0_dout;
      | -- 'TRIG_OUT_1_CONF_1'
      | sm_TRIG_OUT_1_CONF_1_din     <= sm_TRIG_OUT_1_CONF_1_din_i(32-1 downto 0);
      | sm_TRIG_OUT_1_CONF_1_en      <= sm_TRIG_OUT_1_CONF_1_en_i;
      | gen_sm_TRIG_OUT_1_CONF_1_dout_i: if (32 < C_S_AXI_DATA_WIDTH) generate
      |     sm_TRIG_OUT_1_CONF_1_dout_i(C_S_AXI_DATA_WIDTH-1 downto 32) <= (others => '0');
      | end generate gen_sm_TRIG_OUT_1_CONF_1_dout_i;
      | sm_TRIG_OUT_1_CONF_1_dout_i(32-1 downto 0) <= sm_TRIG_OUT_1_CONF_1_dout;
      | -- 'TRIG_OUT_0_CONF_1'
      | sm_TRIG_OUT_0_CONF_1_din     <= sm_TRIG_OUT_0_CONF_1_din_i(32-1 downto 0);
      | sm_TRIG_OUT_0_CONF_1_en      <= sm_TRIG_OUT_0_CONF_1_en_i;
      | gen_sm_TRIG_OUT_0_CONF_1_dout_i: if (32 < C_S_AXI_DATA_WIDTH) generate
      |     sm_TRIG_OUT_0_CONF_1_dout_i(C_S_AXI_DATA_WIDTH-1 downto 32) <= (others => '0');
      | end generate gen_sm_TRIG_OUT_0_CONF_1_dout_i;
      | sm_TRIG_OUT_0_CONF_1_dout_i(32-1 downto 0) <= sm_TRIG_OUT_0_CONF_1_dout;
      | -- 'RSSI_PKT_DET_DURATIONS'
      | sm_RSSI_PKT_DET_DURATIONS_din     <= sm_RSSI_PKT_DET_DURATIONS_din_i(32-1 downto 0);
      | sm_RSSI_PKT_DET_DURATIONS_en      <= sm_RSSI_PKT_DET_DURATIONS_en_i;
      | gen_sm_RSSI_PKT_DET_DURATIONS_dout_i: if (32 < C_S_AXI_DATA_WIDTH) generate
      |     sm_RSSI_PKT_DET_DURATIONS_dout_i(C_S_AXI_DATA_WIDTH-1 downto 32) <= (others => '0');
      | end generate gen_sm_RSSI_PKT_DET_DURATIONS_dout_i;
      | sm_RSSI_PKT_DET_DURATIONS_dout_i(32-1 downto 0) <= sm_RSSI_PKT_DET_DURATIONS_dout;
      | -- 'RSSI_PKT_DET_THRESHOLDS'
      | sm_RSSI_PKT_DET_THRESHOLDS_din     <= sm_RSSI_PKT_DET_THRESHOLDS_din_i(32-1 downto 0);
      | sm_RSSI_PKT_DET_THRESHOLDS_en      <= sm_RSSI_PKT_DET_THRESHOLDS_en_i;
      | gen_sm_RSSI_PKT_DET_THRESHOLDS_dout_i: if (32 < C_S_AXI_DATA_WIDTH) generate
      |     sm_RSSI_PKT_DET_THRESHOLDS_dout_i(C_S_AXI_DATA_WIDTH-1 downto 32) <= (others => '0');
      | end generate gen_sm_RSSI_PKT_DET_THRESHOLDS_dout_i;
      | sm_RSSI_PKT_DET_THRESHOLDS_dout_i(32-1 downto 0) <= sm_RSSI_PKT_DET_THRESHOLDS_dout;
      | -- 'TRIG_IN_CONF_1'
      | sm_TRIG_IN_CONF_1_din     <= sm_TRIG_IN_CONF_1_din_i(32-1 downto 0);
      | sm_TRIG_IN_CONF_1_en      <= sm_TRIG_IN_CONF_1_en_i;
      | gen_sm_TRIG_IN_CONF_1_dout_i: if (32 < C_S_AXI_DATA_WIDTH) generate
      |     sm_TRIG_IN_CONF_1_dout_i(C_S_AXI_DATA_WIDTH-1 downto 32) <= (others => '0');
      | end generate gen_sm_TRIG_IN_CONF_1_dout_i;
      | sm_TRIG_IN_CONF_1_dout_i(32-1 downto 0) <= sm_TRIG_IN_CONF_1_dout;
      | -- 'From FIFO'
      | -- 'To FIFO'
      | -- 'Shared Memory'
      | -- 'PktOps1'
      | sm_PktOps1_addr <= sm_PktOps1_addr_i(6-1 downto 0);
      | sm_PktOps1_din  <= sm_PktOps1_din_i(32-1 downto 0);
      | gen_sm_PktOps1_dout_i: if (32 < C_S_AXI_DATA_WIDTH) generate
      |     sm_PktOps1_dout_i(C_S_AXI_DATA_WIDTH-1 downto 32) <= (others => '0');
      | end generate gen_sm_PktOps1_dout_i;
      | sm_PktOps1_dout_i(32-1 downto 0) <= sm_PktOps1_dout;
      | sm_PktOps1_we <= sm_PktOps1_we_i;
      | -- 'PktTemplate1'
      | sm_PktTemplate1_addr <= sm_PktTemplate1_addr_i(6-1 downto 0);
      | sm_PktTemplate1_din  <= sm_PktTemplate1_din_i(32-1 downto 0);
      | gen_sm_PktTemplate1_dout_i: if (32 < C_S_AXI_DATA_WIDTH) generate
      |     sm_PktTemplate1_dout_i(C_S_AXI_DATA_WIDTH-1 downto 32) <= (others => '0');
      | end generate gen_sm_PktTemplate1_dout_i;
      | sm_PktTemplate1_dout_i(32-1 downto 0) <= sm_PktTemplate1_dout;
      | sm_PktTemplate1_we <= sm_PktTemplate1_we_i;
      | -- 'PktOps0'
      | sm_PktOps0_addr <= sm_PktOps0_addr_i(6-1 downto 0);
      | sm_PktOps0_din  <= sm_PktOps0_din_i(32-1 downto 0);
      | gen_sm_PktOps0_dout_i: if (32 < C_S_AXI_DATA_WIDTH) generate
      |     sm_PktOps0_dout_i(C_S_AXI_DATA_WIDTH-1 downto 32) <= (others => '0');
      | end generate gen_sm_PktOps0_dout_i;
      | sm_PktOps0_dout_i(32-1 downto 0) <= sm_PktOps0_dout;
      | sm_PktOps0_we <= sm_PktOps0_we_i;
      | -- 'PktTemplate0'
      | sm_PktTemplate0_addr <= sm_PktTemplate0_addr_i(6-1 downto 0);
      | sm_PktTemplate0_din  <= sm_PktTemplate0_din_i(32-1 downto 0);
      | gen_sm_PktTemplate0_dout_i: if (32 < C_S_AXI_DATA_WIDTH) generate
      |     sm_PktTemplate0_dout_i(C_S_AXI_DATA_WIDTH-1 downto 32) <= (others => '0');
      | end generate gen_sm_PktTemplate0_dout_i;
      | sm_PktTemplate0_dout_i(32-1 downto 0) <= sm_PktTemplate0_dout;
      | sm_PktTemplate0_we <= sm_PktTemplate0_we_i;
      | 
      | ReadWriteSelect: process(memmap_state) is begin
      |     if (memmap_state = READ) then
      |         -- 'PktOps1'
      |         sm_PktOps1_addr_i <= read_linear_addr_i;-- 'PktTemplate1'
      |         sm_PktTemplate1_addr_i <= read_linear_addr_i;-- 'PktOps0'
      |         sm_PktOps0_addr_i <= read_linear_addr_i;-- 'PktTemplate0'
      |         sm_PktTemplate0_addr_i <= read_linear_addr_i;
      |     else
      |         -- 'PktOps1'
      |         sm_PktOps1_addr_i <= write_linear_addr_i;-- 'PktTemplate1'
      |         sm_PktTemplate1_addr_i <= write_linear_addr_i;-- 'PktOps0'
      |         sm_PktOps0_addr_i <= write_linear_addr_i;-- 'PktTemplate0'
      |         sm_PktTemplate0_addr_i <= write_linear_addr_i;
      |     end if;
      | end process ReadWriteSelect;
      | 
      | -----------------------------------------------------------------------------
      | -- address for 'Shared Memory'
      | -----------------------------------------------------------------------------
      | SharedMemory_Addr_ResetN : process(AXI_AClk) is begin
      |     if (AXI_AClk'event and AXI_AClk = '1') then
      |         if (AXI_AResetN = '0') then
      |             memmap_state <= READ;
      |         else
      |             if (S_AXI_AWVALID = '1') then
      |                 -- write operation
      |                 memmap_state <= WRITE;
      |             elsif (S_AXI_ARVALID = '1') then
      |                 -- read operation
      |                 memmap_state <= READ;
      |             end if;
      |         end if;
      |     end if;
      | end process SharedMemory_Addr_ResetN;
      | 
      | -----------------------------------------------------------------------------
      | -- WRITE Command Control
      | -----------------------------------------------------------------------------
      | S_AXI_BID     <= S_AXI_BID_i;
      | S_AXI_BVALID  <= S_AXI_BVALID_i;
      | S_AXI_WREADY  <= S_AXI_WREADY_i;
      | -- No error checking
      | S_AXI_BRESP  <= (others=>'0');
      | 
      | PROC_AWREADY_ACK: process(read_state, write_state, S_AXI_ARVALID, S_AXI_AWVALID) is begin
      |     if (write_state = IDLE and S_AXI_AWVALID = '1' and read_state = IDLE) then
      |         S_AXI_AWREADY <= S_AXI_AWVALID;
      |     else
      |         S_AXI_AWREADY <= '0';
      |     end if;
      | end process PROC_AWREADY_ACK;
      | 
      | Cmd_Decode_Write: process(AXI_AClk) is begin
      |     if (AXI_AClk'event and AXI_AClk = '1') then
      |         if (AXI_AResetN = '0') then
      |             write_addr_valid    <= '0';
      |             write_ready         <= '0';
      |             s_fifo_we           <= '0';
      |             S_AXI_BVALID_i      <= '0';
      |             S_AXI_BID_i         <= (others => '0');
      |             write_bank_addr_i   <= (others => '0');
      |             write_linear_addr_i <= (others => '0');
      |         else
      |             if (write_state = IDLE) then
      |                 if (S_AXI_AWVALID = '1' and read_state = IDLE) then
      |                     -- reflect awid
      |                     S_AXI_BID_i <= S_AXI_AWID;
      | 
      |                     -- latch bank and linear addresses
      |                     write_bank_addr_i   <= S_AXI_AWADDR(C_S_AXI_TOTAL_ADDR_LEN-1 downto C_S_AXI_LINEAR_ADDR_LEN+2);
      |                     write_linear_addr_i <= S_AXI_AWADDR(C_S_AXI_LINEAR_ADDR_LEN+1 downto 2);
      |                     write_addr_valid <= '1';
      |                     s_fifo_we <= '1';
      | 
      |                     -- write state transition
      |                     write_state <= WRITE_DATA;
      |                 end if;
      |             elsif (write_state = WRITE_DATA) then
      |                 write_ready <= '1';
      |                 s_fifo_we <= '0';
      |                 write_addr_valid <= S_AXI_WVALID;
      |                 
      |                 if (S_AXI_WVALID = '1' and write_ready = '1') then
      |                     write_linear_addr_i <= Std_Logic_Vector(unsigned(write_linear_addr_i) + 1);
      |                 end if;
      | 
      |                 if (S_AXI_WLAST = '1' and write_ready = '1') then
      |                     -- start responding through B channel upon the last write data sample
      |                     S_AXI_BVALID_i <= '1';
      |                     -- write data is over
      |                     write_addr_valid <= '0';
      |                     write_ready <= '0';
      |                     -- write state transition
      |                     write_state <= WRITE_RESPONSE;
      |                 end if;
      |             elsif (write_state = WRITE_RESPONSE) then
      | 
      |                 if (S_AXI_BREADY = '1') then
      |                     -- write respond is over
      |                     S_AXI_BVALID_i <= '0';
      |                     S_AXI_BID_i <= (others => '0');
      | 
      |                     -- write state transition
      |                     write_state <= IDLE;
      |                 end if;
      |             end if;
      |         end if;
      |     end if;
      | end process Cmd_Decode_Write;
      | 
      | Write_Linear_Addr_Decode : process(AXI_AClk) is 
      | 
      | begin
      |     if (AXI_AClk'event and AXI_AClk = '1') then
      |         if (AXI_AResetN = '0') then
      |             -- 'To Register'
      |             -- TRIG_ODELAY_CFG_CMPLL din/en
      |             sm_TRIG_ODELAY_CFG_CMPLL_din_i <= (others => '0');
      |             sm_TRIG_ODELAY_CFG_CMPLL_en_i <= '0';
      |             -- TRIG_IDELAY_CFG_CMPLL din/en
      |             sm_TRIG_IDELAY_CFG_CMPLL_din_i <= (others => '0');
      |             sm_TRIG_IDELAY_CFG_CMPLL_en_i <= '0';
      |             -- TRIG_ODELAY_CFG_DEBUG_HDR din/en
      |             sm_TRIG_ODELAY_CFG_DEBUG_HDR_din_i <= (others => '0');
      |             sm_TRIG_ODELAY_CFG_DEBUG_HDR_en_i <= '0';
      |             -- TRIG_IDELAY_CFG_DEBUG_HDR din/en
      |             sm_TRIG_IDELAY_CFG_DEBUG_HDR_din_i <= (others => '0');
      |             sm_TRIG_IDELAY_CFG_DEBUG_HDR_en_i <= '0';
      |             -- TRIG_IODELAYS_CONTROL din/en
      |             sm_TRIG_IODELAYS_CONTROL_din_i <= (others => '0');
      |             sm_TRIG_IODELAYS_CONTROL_en_i <= '0';
      |             -- RSSI_PKT_DET_CONFIG din/en
      |             sm_RSSI_PKT_DET_CONFIG_din_i <= (others => '0');
      |             sm_RSSI_PKT_DET_CONFIG_en_i <= '0';
      |             -- TRIG_IN_CONF_6 din/en
      |             sm_TRIG_IN_CONF_6_din_i <= (others => '0');
      |             sm_TRIG_IN_CONF_6_en_i <= '0';
      |             -- TRIG_IN_CONF_5 din/en
      |             sm_TRIG_IN_CONF_5_din_i <= (others => '0');
      |             sm_TRIG_IN_CONF_5_en_i <= '0';
      |             -- TRIG_IN_CONF_4 din/en
      |             sm_TRIG_IN_CONF_4_din_i <= (others => '0');
      |             sm_TRIG_IN_CONF_4_en_i <= '0';
      |             -- TRIG_IN_CONF_3 din/en
      |             sm_TRIG_IN_CONF_3_din_i <= (others => '0');
      |             sm_TRIG_IN_CONF_3_en_i <= '0';
      |             -- TRIG_IN_CONF_2 din/en
      |             sm_TRIG_IN_CONF_2_din_i <= (others => '0');
      |             sm_TRIG_IN_CONF_2_en_i <= '0';
      |             -- TRIG_IN_CONF_0 din/en
      |             sm_TRIG_IN_CONF_0_din_i <= (others => '0');
      |             sm_TRIG_IN_CONF_0_en_i <= '0';
      |             -- TRIG_IN_CONF_8 din/en
      |             sm_TRIG_IN_CONF_8_din_i <= (others => '0');
      |             sm_TRIG_IN_CONF_8_en_i <= '0';
      |             -- TRIG_IN_CONF_7 din/en
      |             sm_TRIG_IN_CONF_7_din_i <= (others => '0');
      |             sm_TRIG_IN_CONF_7_en_i <= '0';
      |             -- TRIG_OUT_5_CONF_0 din/en
      |             sm_TRIG_OUT_5_CONF_0_din_i <= (others => '0');
      |             sm_TRIG_OUT_5_CONF_0_en_i <= '0';
      |             -- TRIG_OUT_5_CONF_1 din/en
      |             sm_TRIG_OUT_5_CONF_1_din_i <= (others => '0');
      |             sm_TRIG_OUT_5_CONF_1_en_i <= '0';
      |             -- TRIG_OUT_4_CONF_0 din/en
      |             sm_TRIG_OUT_4_CONF_0_din_i <= (others => '0');
      |             sm_TRIG_OUT_4_CONF_0_en_i <= '0';
      |             -- TRIG_OUT_0_CONF_0 din/en
      |             sm_TRIG_OUT_0_CONF_0_din_i <= (others => '0');
      |             sm_TRIG_OUT_0_CONF_0_en_i <= '0';
      |             -- TRIG_OUT_4_CONF_1 din/en
      |             sm_TRIG_OUT_4_CONF_1_din_i <= (others => '0');
      |             sm_TRIG_OUT_4_CONF_1_en_i <= '0';
      |             -- TRIG_OUT_3_CONF_0 din/en
      |             sm_TRIG_OUT_3_CONF_0_din_i <= (others => '0');
      |             sm_TRIG_OUT_3_CONF_0_en_i <= '0';
      |             -- TRIG_OUT_3_CONF_1 din/en
      |             sm_TRIG_OUT_3_CONF_1_din_i <= (others => '0');
      |             sm_TRIG_OUT_3_CONF_1_en_i <= '0';
      |             -- TRIG_OUT_2_CONF_0 din/en
      |             sm_TRIG_OUT_2_CONF_0_din_i <= (others => '0');
      |             sm_TRIG_OUT_2_CONF_0_en_i <= '0';
      |             -- TRIG_OUT_2_CONF_1 din/en
      |             sm_TRIG_OUT_2_CONF_1_din_i <= (others => '0');
      |             sm_TRIG_OUT_2_CONF_1_en_i <= '0';
      |             -- TRIG_OUT_1_CONF_0 din/en
      |             sm_TRIG_OUT_1_CONF_0_din_i <= (others => '0');
      |             sm_TRIG_OUT_1_CONF_0_en_i <= '0';
      |             -- TRIG_OUT_1_CONF_1 din/en
      |             sm_TRIG_OUT_1_CONF_1_din_i <= (others => '0');
      |             sm_TRIG_OUT_1_CONF_1_en_i <= '0';
      |             -- TRIG_OUT_0_CONF_1 din/en
      |             sm_TRIG_OUT_0_CONF_1_din_i <= (others => '0');
      |             sm_TRIG_OUT_0_CONF_1_en_i <= '0';
      |             -- RSSI_PKT_DET_DURATIONS din/en
      |             sm_RSSI_PKT_DET_DURATIONS_din_i <= (others => '0');
      |             sm_RSSI_PKT_DET_DURATIONS_en_i <= '0';
      |             -- RSSI_PKT_DET_THRESHOLDS din/en
      |             sm_RSSI_PKT_DET_THRESHOLDS_din_i <= (others => '0');
      |             sm_RSSI_PKT_DET_THRESHOLDS_en_i <= '0';
      |             -- TRIG_IN_CONF_1 din/en
      |             sm_TRIG_IN_CONF_1_din_i <= (others => '0');
      |             sm_TRIG_IN_CONF_1_en_i <= '0';
      |             -- 'To FIFO'
      |             -- 'Shared Memory'
      |             -- PktOps1 we
      |             sm_PktOps1_we_i <= '0';
      |             -- PktTemplate1 we
      |             sm_PktTemplate1_we_i <= '0';
      |             -- PktOps0 we
      |             sm_PktOps0_we_i <= '0';
      |             -- PktTemplate0 we
      |             sm_PktTemplate0_we_i <= '0';
      |         else
      |             -- default assignments
      |             -- PktOps1 we
      |             sm_PktOps1_we_i <= '0';
      |             -- PktTemplate1 we
      |             sm_PktTemplate1_we_i <= '0';
      |             -- PktOps0 we
      |             sm_PktOps0_we_i <= '0';
      |             -- PktTemplate0 we
      |             sm_PktTemplate0_we_i <= '0';
      | 
      |             -- 'To Register'
      |             if (unsigned(write_bank_addr_i) = 2) then
      |                 if (unsigned(write_linear_addr_i) = 0) then
      |                     -- TRIG_ODELAY_CFG_CMPLL din/en
      |                     sm_TRIG_ODELAY_CFG_CMPLL_din_i <= S_AXI_WDATA;
      |                     sm_TRIG_ODELAY_CFG_CMPLL_en_i  <= write_addr_valid;
      |                 elsif (unsigned(write_linear_addr_i) = 1) then
      |                     -- TRIG_IDELAY_CFG_CMPLL din/en
      |                     sm_TRIG_IDELAY_CFG_CMPLL_din_i <= S_AXI_WDATA;
      |                     sm_TRIG_IDELAY_CFG_CMPLL_en_i  <= write_addr_valid;
      |                 elsif (unsigned(write_linear_addr_i) = 2) then
      |                     -- TRIG_ODELAY_CFG_DEBUG_HDR din/en
      |                     sm_TRIG_ODELAY_CFG_DEBUG_HDR_din_i <= S_AXI_WDATA;
      |                     sm_TRIG_ODELAY_CFG_DEBUG_HDR_en_i  <= write_addr_valid;
      |                 elsif (unsigned(write_linear_addr_i) = 3) then
      |                     -- TRIG_IDELAY_CFG_DEBUG_HDR din/en
      |                     sm_TRIG_IDELAY_CFG_DEBUG_HDR_din_i <= S_AXI_WDATA;
      |                     sm_TRIG_IDELAY_CFG_DEBUG_HDR_en_i  <= write_addr_valid;
      |                 elsif (unsigned(write_linear_addr_i) = 4) then
      |                     -- TRIG_IODELAYS_CONTROL din/en
      |                     sm_TRIG_IODELAYS_CONTROL_din_i <= S_AXI_WDATA;
      |                     sm_TRIG_IODELAYS_CONTROL_en_i  <= write_addr_valid;
      |                 elsif (unsigned(write_linear_addr_i) = 5) then
      |                     -- RSSI_PKT_DET_CONFIG din/en
      |                     sm_RSSI_PKT_DET_CONFIG_din_i <= S_AXI_WDATA;
      |                     sm_RSSI_PKT_DET_CONFIG_en_i  <= write_addr_valid;
      |                 elsif (unsigned(write_linear_addr_i) = 6) then
      |                     -- TRIG_IN_CONF_6 din/en
      |                     sm_TRIG_IN_CONF_6_din_i <= S_AXI_WDATA;
      |                     sm_TRIG_IN_CONF_6_en_i  <= write_addr_valid;
      |                 elsif (unsigned(write_linear_addr_i) = 7) then
      |                     -- TRIG_IN_CONF_5 din/en
      |                     sm_TRIG_IN_CONF_5_din_i <= S_AXI_WDATA;
      |                     sm_TRIG_IN_CONF_5_en_i  <= write_addr_valid;
      |                 elsif (unsigned(write_linear_addr_i) = 8) then
      |                     -- TRIG_IN_CONF_4 din/en
      |                     sm_TRIG_IN_CONF_4_din_i <= S_AXI_WDATA;
      |                     sm_TRIG_IN_CONF_4_en_i  <= write_addr_valid;
      |                 elsif (unsigned(write_linear_addr_i) = 9) then
      |                     -- TRIG_IN_CONF_3 din/en
      |                     sm_TRIG_IN_CONF_3_din_i <= S_AXI_WDATA;
      |                     sm_TRIG_IN_CONF_3_en_i  <= write_addr_valid;
      |                 elsif (unsigned(write_linear_addr_i) = 10) then
      |                     -- TRIG_IN_CONF_2 din/en
      |                     sm_TRIG_IN_CONF_2_din_i <= S_AXI_WDATA;
      |                     sm_TRIG_IN_CONF_2_en_i  <= write_addr_valid;
      |                 elsif (unsigned(write_linear_addr_i) = 11) then
      |                     -- TRIG_IN_CONF_0 din/en
      |                     sm_TRIG_IN_CONF_0_din_i <= S_AXI_WDATA;
      |                     sm_TRIG_IN_CONF_0_en_i  <= write_addr_valid;
      |                 elsif (unsigned(write_linear_addr_i) = 12) then
      |                     -- TRIG_IN_CONF_8 din/en
      |                     sm_TRIG_IN_CONF_8_din_i <= S_AXI_WDATA;
      |                     sm_TRIG_IN_CONF_8_en_i  <= write_addr_valid;
      |                 elsif (unsigned(write_linear_addr_i) = 13) then
      |                     -- TRIG_IN_CONF_7 din/en
      |                     sm_TRIG_IN_CONF_7_din_i <= S_AXI_WDATA;
      |                     sm_TRIG_IN_CONF_7_en_i  <= write_addr_valid;
      |                 elsif (unsigned(write_linear_addr_i) = 14) then
      |                     -- TRIG_OUT_5_CONF_0 din/en
      |                     sm_TRIG_OUT_5_CONF_0_din_i <= S_AXI_WDATA;
      |                     sm_TRIG_OUT_5_CONF_0_en_i  <= write_addr_valid;
      |                 elsif (unsigned(write_linear_addr_i) = 15) then
      |                     -- TRIG_OUT_5_CONF_1 din/en
      |                     sm_TRIG_OUT_5_CONF_1_din_i <= S_AXI_WDATA;
      |                     sm_TRIG_OUT_5_CONF_1_en_i  <= write_addr_valid;
      |                 elsif (unsigned(write_linear_addr_i) = 16) then
      |                     -- TRIG_OUT_4_CONF_0 din/en
      |                     sm_TRIG_OUT_4_CONF_0_din_i <= S_AXI_WDATA;
      |                     sm_TRIG_OUT_4_CONF_0_en_i  <= write_addr_valid;
      |                 elsif (unsigned(write_linear_addr_i) = 17) then
      |                     -- TRIG_OUT_0_CONF_0 din/en
      |                     sm_TRIG_OUT_0_CONF_0_din_i <= S_AXI_WDATA;
      |                     sm_TRIG_OUT_0_CONF_0_en_i  <= write_addr_valid;
      |                 elsif (unsigned(write_linear_addr_i) = 18) then
      |                     -- TRIG_OUT_4_CONF_1 din/en
      |                     sm_TRIG_OUT_4_CONF_1_din_i <= S_AXI_WDATA;
      |                     sm_TRIG_OUT_4_CONF_1_en_i  <= write_addr_valid;
      |                 elsif (unsigned(write_linear_addr_i) = 19) then
      |                     -- TRIG_OUT_3_CONF_0 din/en
      |                     sm_TRIG_OUT_3_CONF_0_din_i <= S_AXI_WDATA;
      |                     sm_TRIG_OUT_3_CONF_0_en_i  <= write_addr_valid;
      |                 elsif (unsigned(write_linear_addr_i) = 20) then
      |                     -- TRIG_OUT_3_CONF_1 din/en
      |                     sm_TRIG_OUT_3_CONF_1_din_i <= S_AXI_WDATA;
      |                     sm_TRIG_OUT_3_CONF_1_en_i  <= write_addr_valid;
      |                 elsif (unsigned(write_linear_addr_i) = 21) then
      |                     -- TRIG_OUT_2_CONF_0 din/en
      |                     sm_TRIG_OUT_2_CONF_0_din_i <= S_AXI_WDATA;
      |                     sm_TRIG_OUT_2_CONF_0_en_i  <= write_addr_valid;
      |                 elsif (unsigned(write_linear_addr_i) = 22) then
      |                     -- TRIG_OUT_2_CONF_1 din/en
      |                     sm_TRIG_OUT_2_CONF_1_din_i <= S_AXI_WDATA;
      |                     sm_TRIG_OUT_2_CONF_1_en_i  <= write_addr_valid;
      |                 elsif (unsigned(write_linear_addr_i) = 23) then
      |                     -- TRIG_OUT_1_CONF_0 din/en
      |                     sm_TRIG_OUT_1_CONF_0_din_i <= S_AXI_WDATA;
      |                     sm_TRIG_OUT_1_CONF_0_en_i  <= write_addr_valid;
      |                 elsif (unsigned(write_linear_addr_i) = 24) then
      |                     -- TRIG_OUT_1_CONF_1 din/en
      |                     sm_TRIG_OUT_1_CONF_1_din_i <= S_AXI_WDATA;
      |                     sm_TRIG_OUT_1_CONF_1_en_i  <= write_addr_valid;
      |                 elsif (unsigned(write_linear_addr_i) = 25) then
      |                     -- TRIG_OUT_0_CONF_1 din/en
      |                     sm_TRIG_OUT_0_CONF_1_din_i <= S_AXI_WDATA;
      |                     sm_TRIG_OUT_0_CONF_1_en_i  <= write_addr_valid;
      |                 elsif (unsigned(write_linear_addr_i) = 26) then
      |                     -- RSSI_PKT_DET_DURATIONS din/en
      |                     sm_RSSI_PKT_DET_DURATIONS_din_i <= S_AXI_WDATA;
      |                     sm_RSSI_PKT_DET_DURATIONS_en_i  <= write_addr_valid;
      |                 elsif (unsigned(write_linear_addr_i) = 27) then
      |                     -- RSSI_PKT_DET_THRESHOLDS din/en
      |                     sm_RSSI_PKT_DET_THRESHOLDS_din_i <= S_AXI_WDATA;
      |                     sm_RSSI_PKT_DET_THRESHOLDS_en_i  <= write_addr_valid;
      |                 elsif (unsigned(write_linear_addr_i) = 28) then
      |                     -- TRIG_IN_CONF_1 din/en
      |                     sm_TRIG_IN_CONF_1_din_i <= S_AXI_WDATA;
      |                     sm_TRIG_IN_CONF_1_en_i  <= write_addr_valid;
      |                 end if;
      |             end if;        
      |         
      |             -- 'Shared Memory'
      |             if unsigned(write_bank_addr_i) = 0 then
      |                 if (unsigned(write_linear_addr_i(C_S_AXI_LINEAR_ADDR_LEN-1 downto 6)) = 0) then
      |                     -- PktOps1 we
      |                     sm_PktOps1_we_i  <= write_addr_valid;
      |                 elsif (unsigned(write_linear_addr_i(C_S_AXI_LINEAR_ADDR_LEN-1 downto 6)) = 1) then
      |                     -- PktTemplate1 we
      |                     sm_PktTemplate1_we_i  <= write_addr_valid;
      |                 elsif (unsigned(write_linear_addr_i(C_S_AXI_LINEAR_ADDR_LEN-1 downto 6)) = 2) then
      |                     -- PktOps0 we
      |                     sm_PktOps0_we_i  <= write_addr_valid;
      |                 elsif (unsigned(write_linear_addr_i(C_S_AXI_LINEAR_ADDR_LEN-1 downto 6)) = 3) then
      |                     -- PktTemplate0 we
      |                     sm_PktTemplate0_we_i  <= write_addr_valid;
      |                 end if;
      |             end if;        
      |         end if;
      |     end if;
      | end process Write_Linear_Addr_Decode;
      |  
      | -----------------------------------------------------------------------------
      | -- READ Control
      | -----------------------------------------------------------------------------
      | 
      | S_AXI_RDATA  <= S_AXI_RDATA_i;
      | S_AXI_RVALID  <= S_AXI_RVALID_i;
      | S_AXI_RLAST   <= S_AXI_RLAST_i;
      | S_AXI_RID     <= S_AXI_RID_i;
      | -- TODO: no error checking
      | S_AXI_RRESP <= (others=>'0');
      | 
      | PROC_ARREADY_ACK: process(read_state, S_AXI_ARVALID, write_state, S_AXI_AWVALID) is begin
      |     -- Note: WRITE has higher priority than READ
      |     if (read_state = IDLE and S_AXI_ARVALID = '1' and write_state = IDLE and S_AXI_AWVALID /= '1') then
      |         S_AXI_ARREADY <= S_AXI_ARVALID;
      |     else
      |         S_AXI_ARREADY <= '0';
      |     end if;
      | end process PROC_ARREADY_ACK;
      | 
      | S_AXI_WREADY_i <= write_ready;
      | 
      | Process_Sideband: process(write_state, read_state) is begin
      |     if (read_state = READ_PREP) then
      |         s_shram_en <= '1';
      |     elsif (read_state = READ_DATA) then
      |         s_shram_en <= S_AXI_RREADY;
      |     elsif (write_state = WRITE_DATA) then
      |         s_shram_en <= S_AXI_WVALID;
      |     else
      |         s_shram_en <= '0';
      |     end if;
      | end process Process_Sideband;
      | 
      | Cmd_Decode_Read: process(AXI_AClk) is begin
      |     if (AXI_AClk'event and AXI_AClk = '1') then
      |         if (AXI_AResetN = '0') then
      |             S_AXI_RVALID_i <= '0';
      |             read_bank_addr_i    <= (others => '0');
      |             read_linear_addr_i  <= (others => '0');
      |             S_AXI_ARLEN_i       <= (others => '0');
      |             S_AXI_RLAST_i       <= '0';
      |             S_AXI_RID_i         <= (others => '0');
      |             read_state          <= IDLE;
      |             read_prep_counter   <= (others => '0');
      |             read_addr_counter   <= (others => '0');
      |             read_data_counter   <= (others => '0');
      |         else
      |             -- default assignments
      |             s_fifo_re <= '0';
      | 
      |             if (read_state = IDLE) then
      |                 -- Note WRITE has higher priority than READ
      |                 if (S_AXI_ARVALID = '1' and write_state = IDLE and S_AXI_AWVALID /= '1') then
      |                     -- extract bank and linear addresses
      |                     read_bank_addr_i    <= S_AXI_ARADDR(C_S_AXI_TOTAL_ADDR_LEN-1 downto C_S_AXI_LINEAR_ADDR_LEN+2);
      |                     read_linear_addr_i  <= S_AXI_ARADDR(C_S_AXI_LINEAR_ADDR_LEN+1 downto 2);
      |                     s_fifo_re <= '1';
      | 
      |                     -- reflect arid
      |                     S_AXI_RID_i <= S_AXI_ARID;
      | 
      |                     -- load read liner address and data counter
      |                     read_addr_counter <= S_AXI_ARLEN;
      |                     read_data_counter <= S_AXI_ARLEN;
      | 
      |                     -- load read preparation counter
      |                     read_prep_counter <= C_READ_PREP_DELAY;
      |                     -- read state transition
      |                     read_state <= READ_PREP;
      |                 end if;
      |             elsif (read_state = READ_PREP) then
      |                 if (unsigned(read_prep_counter) = 0) then
      |                     if (unsigned(read_data_counter) = 0) then
      |                         -- tag the last data generated by the slave
      |                         S_AXI_RLAST_i <= '1';
      |                     end if;
      |                     -- valid data appears
      |                     S_AXI_RVALID_i <= '1';
      |                     -- read state transition
      |                     read_state <= READ_DATA;
      |                 else
      |                     -- decrease read preparation counter
      |                     read_prep_counter <= Std_Logic_Vector(unsigned(read_prep_counter) - 1);
      |                 end if;
      | 
      |                 if (unsigned(read_prep_counter) /= 3 and unsigned(read_addr_counter) /= 0) then
      |                     -- decrease address counter
      |                     read_addr_counter <= Std_Logic_Vector(unsigned(read_addr_counter) - 1);
      |                     -- increase linear address (no band crossing)
      |                     read_linear_addr_i <= Std_Logic_Vector(unsigned(read_linear_addr_i) + 1);
      |                 end if;
      |             elsif (read_state = READ_DATA) then
      |                 if (S_AXI_RREADY = '1') then
      |                     if (unsigned(read_data_counter) = 1) then
      |                         -- tag the last data generated by the slave
      |                         S_AXI_RLAST_i <= '1';
      |                     end if;
      | 
      |                     if (unsigned(read_data_counter) = 0) then
      |                         -- arid
      |                         S_AXI_RID_i <= (others => '0');
      |                         -- rlast
      |                         S_AXI_RLAST_i <= '0';
      |                         -- no more valid data
      |                         S_AXI_RVALID_i <= '0';
      |                         -- read state transition
      |                         read_state <= IDLE;
      |                     else
      |                         -- decrease read preparation counter
      |                         read_data_counter <= Std_Logic_Vector(unsigned(read_data_counter) - 1);
      | 
      |                         if (unsigned(read_addr_counter) /= 0) then
      |                             -- decrease address counter
      |                             read_addr_counter <= Std_Logic_Vector(unsigned(read_addr_counter) - 1);
      |                             -- increase linear address (no band crossing)
      |                             read_linear_addr_i <= Std_Logic_Vector(unsigned(read_linear_addr_i) + 1);
      |                         end if;
      |                     end if;
      |                 end if;
      |             end if;
      | 
      |         end if;
      |     end if;
      | end process Cmd_Decode_Read;
      | 
      | Read_Linear_Addr_Decode : process(AXI_AClk) is begin
      |     if (AXI_AClk'event and AXI_AClk = '1') then
      |         if (AXI_AResetN = '0') then
      |             reg_bank_out_i   <= (others => '0');
      |             fifo_bank_out_i  <= (others => '0');
      |             shmem_bank_out_i <= (others => '0');
      |             S_AXI_RDATA_i    <= (others => '0');
      |         else
      |             if (unsigned(read_bank_addr_i) = 2) then
      |                 -- 'From Register'
      |                 if (unsigned(read_linear_addr_i) = 29) then
      |                     -- 'CORE_INFO' dout
      |                     reg_bank_out_i <= sm_CORE_INFO_dout_i;
      |                 elsif (unsigned(read_linear_addr_i) = 30) then
      |                     -- 'TRIG_OUT' dout
      |                     reg_bank_out_i <= sm_TRIG_OUT_dout_i;
      |                 end if;
      |                 -- 'To Register' (with register readback)
      |                 if (unsigned(read_linear_addr_i) = 0) then
      |                     -- 'TRIG_ODELAY_CFG_CMPLL' dout
      |                     reg_bank_out_i <= sm_TRIG_ODELAY_CFG_CMPLL_dout_i;
      |                 elsif (unsigned(read_linear_addr_i) = 1) then
      |                     -- 'TRIG_IDELAY_CFG_CMPLL' dout
      |                     reg_bank_out_i <= sm_TRIG_IDELAY_CFG_CMPLL_dout_i;
      |                 elsif (unsigned(read_linear_addr_i) = 2) then
      |                     -- 'TRIG_ODELAY_CFG_DEBUG_HDR' dout
      |                     reg_bank_out_i <= sm_TRIG_ODELAY_CFG_DEBUG_HDR_dout_i;
      |                 elsif (unsigned(read_linear_addr_i) = 3) then
      |                     -- 'TRIG_IDELAY_CFG_DEBUG_HDR' dout
      |                     reg_bank_out_i <= sm_TRIG_IDELAY_CFG_DEBUG_HDR_dout_i;
      |                 elsif (unsigned(read_linear_addr_i) = 4) then
      |                     -- 'TRIG_IODELAYS_CONTROL' dout
      |                     reg_bank_out_i <= sm_TRIG_IODELAYS_CONTROL_dout_i;
      |                 elsif (unsigned(read_linear_addr_i) = 5) then
      |                     -- 'RSSI_PKT_DET_CONFIG' dout
      |                     reg_bank_out_i <= sm_RSSI_PKT_DET_CONFIG_dout_i;
      |                 elsif (unsigned(read_linear_addr_i) = 6) then
      |                     -- 'TRIG_IN_CONF_6' dout
      |                     reg_bank_out_i <= sm_TRIG_IN_CONF_6_dout_i;
      |                 elsif (unsigned(read_linear_addr_i) = 7) then
      |                     -- 'TRIG_IN_CONF_5' dout
      |                     reg_bank_out_i <= sm_TRIG_IN_CONF_5_dout_i;
      |                 elsif (unsigned(read_linear_addr_i) = 8) then
      |                     -- 'TRIG_IN_CONF_4' dout
      |                     reg_bank_out_i <= sm_TRIG_IN_CONF_4_dout_i;
      |                 elsif (unsigned(read_linear_addr_i) = 9) then
      |                     -- 'TRIG_IN_CONF_3' dout
      |                     reg_bank_out_i <= sm_TRIG_IN_CONF_3_dout_i;
      |                 elsif (unsigned(read_linear_addr_i) = 10) then
      |                     -- 'TRIG_IN_CONF_2' dout
      |                     reg_bank_out_i <= sm_TRIG_IN_CONF_2_dout_i;
      |                 elsif (unsigned(read_linear_addr_i) = 11) then
      |                     -- 'TRIG_IN_CONF_0' dout
      |                     reg_bank_out_i <= sm_TRIG_IN_CONF_0_dout_i;
      |                 elsif (unsigned(read_linear_addr_i) = 12) then
      |                     -- 'TRIG_IN_CONF_8' dout
      |                     reg_bank_out_i <= sm_TRIG_IN_CONF_8_dout_i;
      |                 elsif (unsigned(read_linear_addr_i) = 13) then
      |                     -- 'TRIG_IN_CONF_7' dout
      |                     reg_bank_out_i <= sm_TRIG_IN_CONF_7_dout_i;
      |                 elsif (unsigned(read_linear_addr_i) = 14) then
      |                     -- 'TRIG_OUT_5_CONF_0' dout
      |                     reg_bank_out_i <= sm_TRIG_OUT_5_CONF_0_dout_i;
      |                 elsif (unsigned(read_linear_addr_i) = 15) then
      |                     -- 'TRIG_OUT_5_CONF_1' dout
      |                     reg_bank_out_i <= sm_TRIG_OUT_5_CONF_1_dout_i;
      |                 elsif (unsigned(read_linear_addr_i) = 16) then
      |                     -- 'TRIG_OUT_4_CONF_0' dout
      |                     reg_bank_out_i <= sm_TRIG_OUT_4_CONF_0_dout_i;
      |                 elsif (unsigned(read_linear_addr_i) = 17) then
      |                     -- 'TRIG_OUT_0_CONF_0' dout
      |                     reg_bank_out_i <= sm_TRIG_OUT_0_CONF_0_dout_i;
      |                 elsif (unsigned(read_linear_addr_i) = 18) then
      |                     -- 'TRIG_OUT_4_CONF_1' dout
      |                     reg_bank_out_i <= sm_TRIG_OUT_4_CONF_1_dout_i;
      |                 elsif (unsigned(read_linear_addr_i) = 19) then
      |                     -- 'TRIG_OUT_3_CONF_0' dout
      |                     reg_bank_out_i <= sm_TRIG_OUT_3_CONF_0_dout_i;
      |                 elsif (unsigned(read_linear_addr_i) = 20) then
      |                     -- 'TRIG_OUT_3_CONF_1' dout
      |                     reg_bank_out_i <= sm_TRIG_OUT_3_CONF_1_dout_i;
      |                 elsif (unsigned(read_linear_addr_i) = 21) then
      |                     -- 'TRIG_OUT_2_CONF_0' dout
      |                     reg_bank_out_i <= sm_TRIG_OUT_2_CONF_0_dout_i;
      |                 elsif (unsigned(read_linear_addr_i) = 22) then
      |                     -- 'TRIG_OUT_2_CONF_1' dout
      |                     reg_bank_out_i <= sm_TRIG_OUT_2_CONF_1_dout_i;
      |                 elsif (unsigned(read_linear_addr_i) = 23) then
      |                     -- 'TRIG_OUT_1_CONF_0' dout
      |                     reg_bank_out_i <= sm_TRIG_OUT_1_CONF_0_dout_i;
      |                 elsif (unsigned(read_linear_addr_i) = 24) then
      |                     -- 'TRIG_OUT_1_CONF_1' dout
      |                     reg_bank_out_i <= sm_TRIG_OUT_1_CONF_1_dout_i;
      |                 elsif (unsigned(read_linear_addr_i) = 25) then
      |                     -- 'TRIG_OUT_0_CONF_1' dout
      |                     reg_bank_out_i <= sm_TRIG_OUT_0_CONF_1_dout_i;
      |                 elsif (unsigned(read_linear_addr_i) = 26) then
      |                     -- 'RSSI_PKT_DET_DURATIONS' dout
      |                     reg_bank_out_i <= sm_RSSI_PKT_DET_DURATIONS_dout_i;
      |                 elsif (unsigned(read_linear_addr_i) = 27) then
      |                     -- 'RSSI_PKT_DET_THRESHOLDS' dout
      |                     reg_bank_out_i <= sm_RSSI_PKT_DET_THRESHOLDS_dout_i;
      |                 elsif (unsigned(read_linear_addr_i) = 28) then
      |                     -- 'TRIG_IN_CONF_1' dout
      |                     reg_bank_out_i <= sm_TRIG_IN_CONF_1_dout_i;
      |                 end if;
      | 
      |                 S_AXI_RDATA_i <= reg_bank_out_i;
      |             elsif (unsigned(read_bank_addr_i) = 1) then
      |                 -- 'From FIFO'
      |                 -- 'To FIFO'
      | 
      |                 S_AXI_RDATA_i <= fifo_bank_out_i;
      |             elsif (unsigned(read_bank_addr_i) = 0 and s_shram_en = '1') then
      |                 -- 'Shared Memory'
      |                 if (unsigned(read_linear_addr_i(C_S_AXI_LINEAR_ADDR_LEN-1 downto 6)) = 0) then
      |                     -- 'PktOps1' dout
      |                     shmem_bank_out_i <= sm_PktOps1_dout_i;
      |                 elsif (unsigned(read_linear_addr_i(C_S_AXI_LINEAR_ADDR_LEN-1 downto 6)) = 1) then
      |                     -- 'PktTemplate1' dout
      |                     shmem_bank_out_i <= sm_PktTemplate1_dout_i;
      |                 elsif (unsigned(read_linear_addr_i(C_S_AXI_LINEAR_ADDR_LEN-1 downto 6)) = 2) then
      |                     -- 'PktOps0' dout
      |                     shmem_bank_out_i <= sm_PktOps0_dout_i;
      |                 elsif (unsigned(read_linear_addr_i(C_S_AXI_LINEAR_ADDR_LEN-1 downto 6)) = 3) then
      |                     -- 'PktTemplate0' dout
      |                     shmem_bank_out_i <= sm_PktTemplate0_dout_i;
      |                 end if;
      | 
      |                 S_AXI_RDATA_i <= shmem_bank_out_i;
      |             end if;
      |         end if;
      |     end if;
      | end process Read_Linear_Addr_Decode;
      | 
      | end architecture IMP;
      settings: infoedit=For use with EDK Processor block.
  wires:
  memmap/82 -> Shared Memory3/4, Shared Memory2/4, Shared Memory1/4, Shared Memory/4
  memmap/43 -> To Register15/2
  memmap/42 -> To Register15/1
  memmap/41 -> To Register14/2
  memmap/40 -> To Register14/1
  memmap/49 -> To Register18/2
  memmap/48 -> To Register18/1
  memmap/45 -> To Register16/2
  memmap/44 -> To Register16/1
  memmap/53 -> To Register20/2
  memmap/52 -> To Register20/1
  memmap/51 -> To Register19/2
  memmap/50 -> To Register19/1
  memmap/57 -> To Register22/2
  memmap/56 -> To Register22/1
  memmap/55 -> To Register21/2
  memmap/54 -> To Register21/1
  memmap/61 -> To Register24/2
  memmap/60 -> To Register24/1
  memmap/59 -> To Register23/2
  memmap/58 -> To Register23/1
  memmap/63 -> To Register25/2
  memmap/62 -> To Register25/1
  memmap/47 -> To Register17/2
  memmap/46 -> To Register17/1
  memmap/17 -> To Register2/2
  memmap/16 -> To Register2/1
  memmap/13 -> To Register/2
  memmap/12 -> To Register/1
  memmap/21 -> To Register4/2
  memmap/20 -> To Register4/1
  memmap/37 -> To Register12/2
  memmap/36 -> To Register12/1
  memmap/39 -> To Register13/2
  memmap/38 -> To Register13/1
  memmap/25 -> To Register6/2
  memmap/24 -> To Register6/1
  memmap/27 -> To Register7/2
  memmap/26 -> To Register7/1
  memmap/29 -> To Register8/2
  memmap/28 -> To Register8/1
  memmap/31 -> To Register9/2
  memmap/30 -> To Register9/1
  memmap/33 -> To Register10/2
  memmap/32 -> To Register10/1
  memmap/69 -> To Register28/2
  memmap/68 -> To Register28/1
  memmap/35 -> To Register11/2
  memmap/34 -> To Register11/1
  memmap/19 -> To Register3/2
  memmap/18 -> To Register3/1
  memmap/15 -> To Register1/2
  memmap/14 -> To Register1/1
  memmap/67 -> To Register27/2
  memmap/66 -> To Register27/1
  memmap/65 -> To Register26/2
  memmap/64 -> To Register26/1
  memmap/23 -> To Register5/2
  memmap/22 -> To Register5/1
  memmap/75 -> Shared Memory1/3
  memmap/74 -> Shared Memory1/2
  memmap/73 -> Shared Memory1/1
  memmap/81 -> Shared Memory3/3
  memmap/80 -> Shared Memory3/2
  memmap/79 -> Shared Memory3/1
  memmap/72 -> Shared Memory/3
  memmap/71 -> Shared Memory/2
  memmap/70 -> Shared Memory/1
  memmap/78 -> Shared Memory2/3
  memmap/77 -> Shared Memory2/2
  memmap/76 -> Shared Memory2/1
  memmap/11 -> S_AXI_WREADY/1
  memmap/10 -> S_AXI_RVALID/1
  memmap/9 -> S_AXI_RRESP/1
  memmap/8 -> S_AXI_RLAST/1
  memmap/7 -> S_AXI_RID/1
  memmap/6 -> S_AXI_RDATA/1
  memmap/5 -> S_AXI_BVALID/1
  memmap/4 -> S_AXI_BRESP/1
  memmap/3 -> S_AXI_BID/1
  memmap/2 -> S_AXI_AWREADY/1
  memmap/1 -> S_AXI_ARREADY/1
  S_AXI_WVALID/1 -> memmap/25
  S_AXI_WSTRB/1 -> memmap/24
  S_AXI_WLAST/1 -> memmap/23
  S_AXI_WDATA/1 -> memmap/22
  S_AXI_RREADY/1 -> memmap/21
  S_AXI_BREADY/1 -> memmap/20
  S_AXI_AWVALID/1 -> memmap/19
  S_AXI_AWSIZE/1 -> memmap/18
  S_AXI_AWPROT/1 -> memmap/17
  S_AXI_AWLOCK/1 -> memmap/16
  S_AXI_AWLEN/1 -> memmap/15
  S_AXI_AWID/1 -> memmap/14
  S_AXI_AWCACHE/1 -> memmap/13
  S_AXI_AWBURST/1 -> memmap/12
  S_AXI_AWADDR/1 -> memmap/11
  S_AXI_ARVALID/1 -> memmap/10
  S_AXI_ARSIZE/1 -> memmap/9
  S_AXI_ARPROT/1 -> memmap/8
  S_AXI_ARLOCK/1 -> memmap/7
  S_AXI_ARLEN/1 -> memmap/6
  S_AXI_ARID/1 -> memmap/5
  S_AXI_ARCACHE/1 -> memmap/4
  S_AXI_ARBURST/1 -> memmap/3
  S_AXI_ARADDR/1 -> memmap/2
  AXI_ARESETN/1 -> memmap/1
  From Register1/1 -> memmap/27
  To Register15/1 -> memmap/43
  To Register14/1 -> memmap/42
  To Register18/1 -> memmap/46
  To Register16/1 -> memmap/44
  To Register20/1 -> memmap/48
  To Register19/1 -> memmap/47
  To Register22/1 -> memmap/50
  To Register21/1 -> memmap/49
  To Register24/1 -> memmap/52
  To Register23/1 -> memmap/51
  To Register25/1 -> memmap/53
  To Register17/1 -> memmap/45
  To Register2/1 -> memmap/30
  To Register/1 -> memmap/28
  To Register4/1 -> memmap/32
  To Register12/1 -> memmap/40
  To Register13/1 -> memmap/41
  To Register6/1 -> memmap/34
  To Register7/1 -> memmap/35
  To Register8/1 -> memmap/36
  To Register9/1 -> memmap/37
  To Register10/1 -> memmap/38
  To Register28/1 -> memmap/56
  To Register11/1 -> memmap/39
  To Register3/1 -> memmap/31
  To Register1/1 -> memmap/29
  To Register27/1 -> memmap/55
  To Register26/1 -> memmap/54
  To Register5/1 -> memmap/33
  Shared Memory1/1 -> memmap/58
  Shared Memory3/1 -> memmap/60
  Shared Memory/1 -> memmap/57
  Shared Memory2/1 -> memmap/59
  From Register/1 -> memmap/26
  S_AXI_WREADY/1 -> Terminator10/1
  S_AXI_RVALID/1 -> Terminator9/1
  S_AXI_RRESP/1 -> Terminator8/1
  S_AXI_RLAST/1 -> Terminator7/1
  S_AXI_RID/1 -> Terminator6/1
  S_AXI_RDATA/1 -> Terminator5/1
  S_AXI_BVALID/1 -> Terminator4/1
  S_AXI_BRESP/1 -> Terminator3/1
  S_AXI_BID/1 -> Terminator2/1
  S_AXI_AWREADY/1 -> Terminator1/1
  S_AXI_ARREADY/1 -> Terminator/1
  Constant24/1 -> S_AXI_WVALID/1
  Constant23/1 -> S_AXI_WSTRB/1
  Constant22/1 -> S_AXI_WLAST/1
  Constant21/1 -> S_AXI_WDATA/1
  Constant20/1 -> S_AXI_RREADY/1
  Constant19/1 -> S_AXI_BREADY/1
  Constant18/1 -> S_AXI_AWVALID/1
  Constant17/1 -> S_AXI_AWSIZE/1
  Constant16/1 -> S_AXI_AWPROT/1
  Constant15/1 -> S_AXI_AWLOCK/1
  Constant14/1 -> S_AXI_AWLEN/1
  Constant13/1 -> S_AXI_AWID/1
  Constant12/1 -> S_AXI_AWCACHE/1
  Constant11/1 -> S_AXI_AWBURST/1
  Constant10/1 -> S_AXI_AWADDR/1
  Constant9/1 -> S_AXI_ARVALID/1
  Constant8/1 -> S_AXI_ARSIZE/1
  Constant7/1 -> S_AXI_ARPROT/1
  Constant6/1 -> S_AXI_ARLOCK/1
  Constant5/1 -> S_AXI_ARLEN/1
  Constant4/1 -> S_AXI_ARID/1
  Constant3/1 -> S_AXI_ARCACHE/1
  Constant2/1 -> S_AXI_ARBURST/1
  Constant1/1 -> S_AXI_ARADDR/1
  Constant/1 -> AXI_ARESETN/1
